simulink model "Microgrid_transition_model_113021_ben"  (R2020a)
settings: Solver=VariableStepAuto  StartTime=0.0  StopTime=1  MaxStep=1e-4  RelTol=1e-3
PreLoadFcn:
  | %run('FC_microgrid_param.m')
  | %load('gen_grid_init.mat')
InitFcn:
  | %load myisoModel_init;
  | run('FC_microgrid_param.m')
  | tic
  | run('CARTinitFcn.m')
  | %caseNo = 2;
  | 
  | %if (caseNo == 1)
  | %set_param(['Isolated_grid_paper_model_022521/SignalGen'], 'ActiveScenario', 'PStep222kW');
  | %else
  | %set_param(['Isolated_grid_paper_model_022521/SignalGen'], 'ActiveScenario', 'QStep222kVAr');
  | 
  | %end;
StopFcn:
  | toc
undefined symbols (not defined in the file or in its folder): breakpoints1, breakpoints2, cc_kp, cp_table_data, ctrl, D1, Delta, DiscIntNeverNeededParam, DT, FC_BESS, FC_PV_FirstSolar, find_system, gcbh, libFC_BESS, libFC_PV, LowerLimit, magnitude, oversize, pll_ki, pll_kp, pq_ts, sps_rtmsupport, timer, ts, Ts, Ts_APC, Ts_Control, Ts_Power, UpperLimit
libraries: powerlib x152, powerlib_extras x100, simulink x95, powerlib_meascontrol x90, eePowerMeasurement x40, pi_ctrl x16, simulink_extras x12, sps_avr x7, spsDieselMotorModel x3, libFSArray x2, SignalEditorBlockLib x2, libLgBattery x1
(part 1 of 14)
CloseFcn:
  | toc
settings Model: SimulationMode=accelerator  Creator=rpoudel  LastModifiedBy=banderso2
settings SolverCC: ZeroCrossAlgorithm=Adaptive
settings DataIOCC: SaveOperatingPoint=on  SaveFormat=StructureWithTime  SaveOutput=off  SignalLogging=off  DSMLogging=off  SaveTime=off  ReturnWorkspaceOutputs=off
settings OptimizationCC: EfficientMapNaN2IntZero=off
settings DebuggingCC: IgnoredZcDiagnostic=none  UnconnectedInputMsg=none  UnconnectedOutputMsg=none  UnconnectedLineMsg=none  ArithmeticOperatorsInVariantConditions=warning
settings HardwareCC: TargetBitPerPointer=64  TargetBitPerSizeT=64  TargetBitPerPtrDiffT=64  TargetLongLongMode=on  TargetIntDivRoundTo=Zero  TargetEndianess=LittleEndian  TargetWordSize=64  TargetHWDeviceType=MATLAB Host  ProdEqTarget=off
settings SFSimCC: SimUseLocalCustomCode=off  CustomCodeUndefinedFunction=UseInterfaceOnly
settings RTWCC: SystemTargetFile=accel.tlc  TemplateMakefile=accel_default_tmf  RTWVerbose=off
settings CodeAppCC: MaxIdLength=128
settings STFCustomTargetCC: TargetLangStandard=C99 (ISO)  ConcurrentExecutionCompliant=on  MATLABClassNameForMDSCustomization=Simulink.SoftwareTarget.TargetSpecificTriggerConfigurationBase  GRTInterface=on  SystemTargetFile=accel.tlc

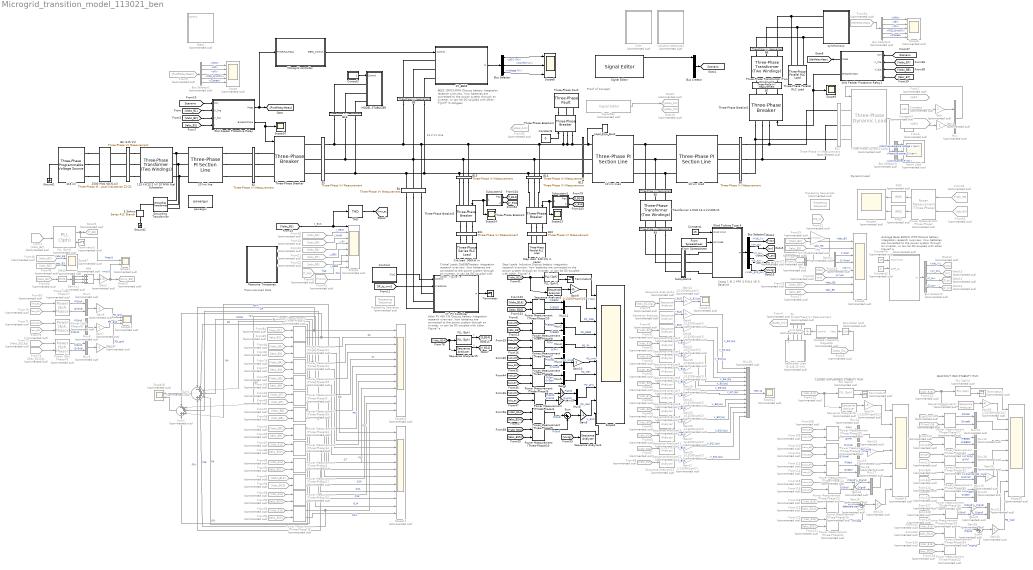
== system Microgrid_transition_model_113021_ben ==
  note: CLOSED UNPLANNED STABILITY RUN
  note: Dynamic Load
  note: Proof of Concept
  note: Critical Loads
      | Discuss battery integration research overview, how batteries are connected to the power system through an inverter, or can be DC-coupled with other. Figure?
      |
      | e
  note: Resource/Load Data
  note: 13.2 kV LIne
  note: Eaton Switchgear
  note: BESS 1MW/1MWh
      | Discuss battery integration research overview, how batteries are connected to the power system through an inverter, or can be DC-coupled with other. Figure?
      |
      | e
  note: Solar PV 430 kW
      | Discuss battery integration research overview, how batteries are connected to the power system through an inverter, or can be DC-coupled with other. Figure?
      |
      | e
  note: Step Loads: Inductive
      | Discuss battery integration research overview, how batteries are connected to the power system through an inverter, or can be DC-coupled with other. Figure?
      |
      | e
  note: Average Base 600kW WTG
      | Discuss battery integration research overview, how batteries are connected to the power system through an inverter, or can be DC-coupled with other. Figure?
      |
      | e
  note: Cases
      | 1 IR
      | 2 PFR
      | 3 P/Q
      | 4 VR
      | 5 Baseline
  note: BLACKOUT GEN STABILITY RUN
  .. : Subsystem  Commented=on  LoadFcn=%find_system(gcs,'FollowLinks', 'on', 'LookUnderMasks', 'all');  mask(Wind Turbine: Model 7){Nb_wt=1, ShowParameters=Drive train data for 1 wind turbine, nom=[6e5/0.9 730 60], Reactances=[ 1.305, 0.296, 0.252, 0.474,  0.243,  0.18 ], Time_constants=[4.49  0.0681  0.0513  ], Resistance=0.006, mec=[0.62/10 0.01 1], init=[ 0  0  0  0  0  0  0  0  1 ], Vnom=575, Imax_grid_conv=1.1, RL_grid=[ 0.15 0.15/50], C_var_filter1=150e3, Vdc_nom=1100, C_DClink1=90000e-6, L_R_Boost=[0.0012     5e-3], Pmec1=6e5, wind_speed_CpMax=11, wind0=11, DisplayTurbChar=off, H_WT=4.32, Ksh=0.0446, D_mutual=1.5, w_wt0=1, torque0=1, Kdc=[1.1   27.5], Ki_var_reg=0.05, Ki_volt_reg=2, Kgrid_side_cur_reg=[1  50], Kspeed=[5 1], Kboost_cur_reg=[0.025 100], Kp_pitch=15, Kcompensation=[1.5  6], Kfield=[10  20], pitch_max=27, pitch_rate=10, Ts=Ts}
      mask prompts: Nb_wt "Number of wind turbines:"; ShowParameters "Display:"; nom "Nom. power, L-L volt. and freq.: [Pn (VA), Vn (Vrms), fn (Hz)]"; Reactances "Reactances [Xd Xd' Xd'' Xq Xq'' Xl] (p.u.):"; Time_constants "Time constants [Tdo' Tdo'' Tq''] (s):"; Resistance "Resistance Rs (p.u.):"; mec "Inertia constant, friction factor, and pairs of poles: [ H(s)  F(p.u.)  p ]"; init "Initial conditions: [dw(%) th(deg) ia,ib,ic(pu) pha,phb,phc(deg) Vf(pu)]:"; Vnom "Grid-side converter nominal AC voltage (V):"; Imax_grid_conv "Grid-side converter maximum AC current (pu based on generator power and converter nominal AC voltage):"; RL_grid "Grid-side coupling inductor [ L(pu) R(pu),pu based on generator power and converter nominal AC voltage] :"; C_var_filter1 "Line filter capacitor (Q=50) (var):"; Vdc_nom "Nominal DC bus voltage (V)"; C_DClink1 "DC bus capacitor (F):"; L_R_Boost "Boost converter inductance [L(H) R(ohm)]:"; Pmec1 "Nominal mechanical output power (W):"; wind_speed_CpMax "Wind speed at nominal speed and at Cp max (must be between 6 m/s and 30 m/s) (m/s):"; wind0 "Initial wind speed (m/s):"; DisplayTurbChar "Display wind turbine power characteristics:"; H_WT "Wind turbine inertia constant H (s):"; Ksh "Shaft spring constant refer to high-speed shaft (pu of nominal mechanical torque/rad):"; D_mutual "Shaft mutual damping (pu of nominal mechanical torque/pu dw):"; w_wt0 "Turbine initial speed (pu of nominal speed):"; torque0 "Initial output torque (pu of nominal mechanical torque):"; Kdc "DC bus voltage regulator gains [Kp Ki]:"; Ki_var_reg "Grid-side converter var regulator gain [ Ki]:"; Ki_volt_reg "Grid-side converter voltage regulator gain [ Ki]:"; Kgrid_side_cur_reg "Grid-side converter current regulator gains [Kp Ki]:"; Kspeed "Speed regulator gains [Kp Ki]:"; Kboost_cur_reg "Boost inductor current regulator gains [Kp Ki]:"; Kp_pitch "Pitch controller gain [Kp]:"; Kcompensation "Pitch compensation gains [Kp Ki]:"; Kfield "Field excitation gains [Kp Ki]:"; pitch_max "Maximum pitch angle (deg):"; pitch_rate "Maximum rate of change of pitch angle (deg/s)"; Ts "Sample time (s):"
      mask help: This block implements a model of a variable speed pitch controlled wind turbine using a synchronous generator.
      mask init:
      | %Generator data
      | Pnom=nom(1)*Nb_wt;
      | Vnom_gen=nom(2);
      | Fnom=nom(3);
      | Xd=Reactances(1);
      | Xd1=Reactances(2);
      | Xd2=Reactances(3);
      | Xq=Reactances(4);
      | Xq2=Reactances(5);
      | Xl=Reactances(6);
      | Tdo1=Time_constants(1);
      | Tdo2=Time_constants(2);
      | Tq2=Time_constants(3);
      | H=mec(1);
      | F=mec(2);
      | p=mec(3);
      | 
      | % Converters data
      | L_RL=RL_grid(1);
      | R_RL=RL_grid(2);
      | L_Boost=L_R_Boost(1)/Nb_wt;
      | R_Boost=L_R_Boost(2)/Nb_wt;
      | Q_filter=50;
      | C_DClink=C_DClink1*Nb_wt;
      | C_var_filter=C_var_filter1*Nb_wt;
      | 
      | % Controller data
      | Freq_filter=10000;   %Hz
      | Zeta_filter=0.707;
      | Kp_dc=Kdc(1);
      | Ki_dc=Kdc(2);
      | Kp_grid_side_cur_reg=Kgrid_side_cur_reg(1);
      | Ki_grid_side_cur_reg=Kgrid_side_cur_reg(2);
      | Kp_speed=Kspeed(1);
      | Ki_speed=Kspeed(2);
      | Kp_boost_cur_reg=Kboost_cur_reg(1);
      | Ki_boost_cur_reg=Kboost_cur_reg(2);
      | Kp_compensation=Kcompensation(1);
      | Ki_compensation=Kcompensation(2);
      | Kp_field=Kfield(1);
      | Ki_field=Kfield(2);
      | Mod_index_max=1.1;
      | T_speed=5;      %Speed reference time constant (s)
      | Iq_ref_limit_time_constant=0.3; %(s)
      | Current_reg_output_limit=1.1;   %(pu)
      | Var_reg_output_hi_limit=1.1;    %(pu)
      | Var_reg_output_low_limit=0.9;   %(pu)
      | Pitch_time_constant=0.01;       %(s)
      | Vf_limit=10;    %Field voltage limit (pu)
      | Flux_meas_time_constant=1*(1/Fnom); %(s)
      | Ts_snub=50e-6;  %Sample time to compute snubber resistance
      | 
      | 
      | % Turbine data
      | Pmec=Pmec1*Nb_wt;
      | c1 = 0.6450;
      | c2 = 116;
      | c3 = .4;
      | c4 = 5;
      | c5 = 21;
      | c6 = .00912;  % Set Pmin in stall condition (does not vary with wind_speed_Pmax)
      | c7 = .08;
      | c8 = .035;
      | theta=0;
      | CpMax=.465;     %.5;
      | lambda_CpMax=6; %9.9495;
      | 
      | c1_c8=[c1 c2 c3 c4 c5 c6 c7 c8];
      |   
      | 
      | %   Cp = c1*(c6*lambda + (-c4 - c3*(2.5 + theta) + c2*(1/(lambda + ...
      | %   c7*(2.5 + theta)) - c8/(1 + (2.5 + theta)^3)))/exp(c5*(1/(lambda + ...
      | %   c7*(2.5 + theta)) - c8/(1 + (2.5 + theta)^3))))
      | 
      | 
      |         %%%%%%%%%%%%%%%%%%%%%%%%%%%%%%%%%%%%%%%%%%%%%%%%%%%%%%%%%%%%%%%%%%%%%%%%%%%
      |         % Operation at Cp max
      |         %%%%%%%%%%%%%%%%%%%%%%%%%%%%%%%%%%%%%%%%%%%%%%%%%%%%%%%%%%%%%%%%%%%%%%%%%%%
      |         
      |         rated_omegar=1;
      |         omegar = rated_omegar;
      |         
      |         % Enforce boundaries on wind speed
      |         % A warning could be displayed
      |         if wind_speed_CpMax < 6
      |             wind_speed_CpMax=6;
      |             disp('Warning: Wind speed at nominal speed and at Cp max has been set to 6 m/s')
      |         end
      |         if wind_speed_CpMax > 30
      |             wind_speed_CpMax=30;
      |             disp('Warning: Wind speed at nominal speed and at Cp max has been set to 30 m/s')
      |         end
      | 
      |         K1=lambda_CpMax/omegar*wind_speed_CpMax;
      |         
      |         % Calculation of K2 needed to get P equal to the requested value at
      |         % Cp max for the requested wind speed
      |         
      |         Prated=Pmec;
      |         P_rated_omegar_theta_zero=1; %0.75;
      |         
      |         K2 = P_rated_omegar_theta_zero*Prated/(wind_speed_CpMax^3*CpMax);
      |         
      |         K1_K2=[K1 K2];
      |         
      |         %%%%%%%%%%%%%%%%%%%%%%%%%%%%%%%%%%%%%%%%%%%%%%%%%%%%%%%%%%%%%%%%%%%%%%%%%%%
      |         % End of calculation for operation at Cp max
      |         %%%%%%%%%%%%%%%%%%%%%%%%%%%%%%%%%%%%%%%%%%%%%%%%%%%%%%%%%%%%%%%%%%%%%%%%%%%
      |         
      | 
      | %%%%%%%%%%%%%%%%%%%%%%%%%%%%%%%%%%%%%%%%%%%%%%%%%%%%%%%%%%%%%%%%%%%%%%%%%%%
      | % Plot turbine characteristics
      | %%%%%%%%%%%%%%%%%%%%%%%%%%%%%%%%%%%%%%%%%%%%%%%%%%%%%%%%%%%%%%%%%%%%%%%%%%% 
      | 
      | DisplayTurbChar=get_param(gcb,'DisplayTurbChar');
      | if strcmp(DisplayTurbChar,'on')
      |     vect_theta = 0:2:30;
      |     
      |     vect_lambda = 1:0.2:30;
      |     
      |     clear Cp;
      |     
      |     for i=1:length(vect_theta)
      |      for j=1:length(vect_lambda)
      |                 Cp(i,j) = c1*(c6*vect_lambda(j) + (-c4 - c3*(2.5 + vect_theta(i)) + c2*(1/(vect_lambda(j) + ...
      |                 c7*(2.5 + vect_theta(i))) - c8/(1 + (2.5 + vect_theta(i))^3)))/exp(c5*(1/(vect_lambda(j) + ...
      |                 c7*(2.5 + vect_theta(i))) - c8/(1 + (2.5 + vect_theta(i))^3))));
      |      end
      |     end
      | 
      |     figure(1);
      |     clf;
      |     hold on;
      | 
      |     plot(vect_lambda, Cp);
      |     axis([0, 25, 0, .6]);
      |     title('Wind Turbine Cp Characteristic (pitch angle increases by step of 2 deg.)');
      |     ylabel('Cp');
      |     set(gca,'ytick',[0 .1 .2 .3 .4 .5 .6]);
      |     xlabel('Lambda');
      |     grid on;
      |     text(10.1,0.51,'Pitch angle 0 degree');
      | 
      |     hold off
      |     
      |     % Plot of the wind turbine mechanical power output (pu) lambda and Cp
      |     % characteristics against wind speed (m/s) for a range of theta.
      |     
      |     wind_speed_range = [1,.2,30];
      |     vect_wind_speed = 1:0.2:30;
      |     
      |     clear lambda;
      |     clear Cp;
      |     clear P;
      | 
      |     for i=1:length(vect_theta)
      |         for j=1:length(vect_wind_speed)
      |             lambda(i,j) = K1*omegar/vect_wind_speed(j);
      |             Cp(i,j) = c1*(c6*lambda(i,j) + (-c4 - c3*(2.5 + vect_theta(i)) + c2*(1/(lambda(i,j) + ...
      |             c7*(2.5 + vect_theta(i))) - c8/(1 + (2.5 + vect_theta(i))^3)))/exp(c5*(1/(lambda(i,j) + ...
      |             c7*(2.5 + vect_theta(i))) - c8/(1 + (2.5 + vect_theta(i))^3))));
      |             P(i,j) = K2/Prated*vect_wind_speed(j)^3*Cp(i,j);
      |         end
      |     end
      |     
      |     
      |     figure(2);
      |     clf;
      |     hold on
      |     
      |     subplot(3,1,1);
      |     plot(vect_wind_speed, P);
      |     axis([0, 35, 0, 1.5]);
      |     title('Wind Turbine Characteristics (w = 1 pu, pitch angle increases by step of 2 deg.)');
      |     ylabel('P (pu)');
      |     set(gca,'ytick',0:.5:4);
      |     grid on;
      |     
      |     subplot(3,1,2);
      |     plot(vect_wind_speed, lambda);
      |     axis([0, 35, 0, 20]);
      |     ylabel('Lambda');
      |     grid on;
      |     
      |     subplot(3,1,3)
      |     plot(vect_wind_speed, Cp);
      |     axis([0, 35, 0, .6]);
      |     xlabel('Wind Speed (m/s)');
      |     ylabel('Cp');
      |     set(gca,'ytick',[0 .1 .2 .3 .4 .5 .6]);
      |     grid on;
      | 
      |     hold off
      |     set_param(gcb,'DisplayTurbChar','off')
      |     
      | end
      mask TypeOptions ShowParameters: Generator data for 1 wind turbine | Converters data for 1 wind turbine | Turbine data for 1 wind turbine | Drive train data for 1 wind turbine | Control parameters for 1 wind turbine
      mask Callback ShowParameters:
      | BlockName=getfullname(gcb);
      | %
      | Param_Show=get_param(BlockName,'ShowParameters');
      | Param_DisplayTurbChar=get_param(BlockName,'DisplayTurbChar');
      | 
      | p_mask{3}='off';p_mask{4}='off';p_mask{5}='off';
      | p_mask{6}='off';p_mask{7}='off';p_mask{8}='off';p_mask{9}='off';
      | p_mask{10}='off';p_mask{11}='off';p_mask{12}='off';p_mask{13}='off';
      | p_mask{14}='off';p_mask{15}='off';p_mask{16}='off';p_mask{17}='off';
      | p_mask{18}='off';p_mask{19}='off';p_mask{20}='off';p_mask{21}='off';
      | p_mask{22}='off';p_mask{23}='off';p_mask{24}='off';p_mask{25}='off';
      | p_mask{26}='off';p_mask{27}='off';p_mask{28}='off';p_mask{29}='off';
      | p_mask{30}='off';p_mask{31}='off';p_mask{32}='off';p_mask{33}='off';
      | p_mask{34}='off';p_mask{35}='off';
      | 
      | switch Param_Show
      | 	case 'Generator data for 1 wind turbine'
      | 		p_mask{3}='on';p_mask{4}='on';p_mask{5}='on';
      |         p_mask{6}='on';p_mask{7}='on';p_mask{8}='on';
      |     case 'Converters data for 1 wind turbine'
      | 		p_mask{9}='on';p_mask{10}='on';p_mask{11}='on';
      |         p_mask{12}='on';p_mask{13}='on';p_mask{14}='on';p_mask{15}='on';
      | 	case 'Turbine data for 1 wind turbine'
      | 		p_mask{16}='on';p_mask{17}='on';p_mask{18}='on';p_mask{19}='on';
      |     case 'Drive train data for 1 wind turbine'
      |         p_mask{20}='on';p_mask{21}='on';p_mask{22}='on';p_mask{23}='on';
      |         p_mask{24}='on';
      |     case 'Control parameters for 1 wind turbine'
      |         p_mask{25}='on';p_mask{26}='on';p_mask{27}='on';
      |         p_mask{28}='on';p_mask{29}='on';p_mask{30}='on';p_mask{31}='on';
      |         p_mask{32}='on';p_mask{33}='on';p_mask{34}='on';p_mask{35}='on';
      | end
      | 
      | ParVisible={'on','on',p_mask{3},p_mask{4},p_mask{5},p_mask{6},...
      |     p_mask{7},p_mask{8},p_mask{9},p_mask{10},p_mask{11},p_mask{12},...
      |     p_mask{13},p_mask{14},p_mask{15},p_mask{16},p_mask{17},p_mask{18},...
      |     p_mask{19},p_mask{20},p_mask{21},p_mask{22},p_mask{23},p_mask{24},...
      |     p_mask{25},p_mask{26},p_mask{27},p_mask{28},p_mask{29},p_mask{30},...
      |     p_mask{31},p_mask{32},p_mask{33},p_mask{34},p_mask{35},'on'};
      | %
      | set_param(BlockName,'MaskVisibilities',ParVisible);
      | set_param(BlockName,'DisplayTurbChar',Param_DisplayTurbChar);
      mask Display: image('$imagefile'); % Use "Edit Image" on toolstrip to change.
  10 km line : powerlib/Elements/Three-Phase PI Section Line  LConnTagsString=a|b|c  RConnTagsString=A|B|C  Frequency=60  Resistances=[0.1153 0.413]  Inductances=[1.05e-3 3.32e-3]  Capacitances=[11.33e-009 5.01e-009]  Length=10
  10 km line1 : powerlib/Elements/Three-Phase PI Section Line  LConnTagsString=a|b|c  RConnTagsString=A|B|C  Frequency=60  Resistances=[0.1153 0.413]  Inductances=[1.05e-3 3.32e-3]  Capacitances=[11.33e-009 5.01e-009]  Length=0.1
  10 km line2 : powerlib/Elements/Three-Phase PI Section Line  LConnTagsString=a|b|c  RConnTagsString=A|B|C  Frequency=60  Resistances=[0.1153 0.413]  Inductances=[1.05e-3 3.32e-3]  Capacitances=[11.33e-009 5.01e-009]  Length=0.01
  115 kV : powerlib/Electrical Sources/Three-Phase Programmable Voltage Source  PositiveSequence=[115e3 0 60]  VariationEntity=None  VariationType=Table of time-amplitude pairs  VariationTypeAlt=Step  VariationStep=-0.2  VariationRate=10  VariationMagnitude=0.3  VariationFrequency=2  VariationTiming=[0.05 0.05+5/60]  VariationPhaseA=off  Amplitudes=[1 1 1.0]  TimeValues=[0 0.03 0.13]  HarmonicGeneration=off  HarmonicA=[1 -0.1 0 2]  HarmonicB=[2 0.15 35 2]*0  Timing="[0.1  2]"  BusType=swing  Pref=0  Qref=0  Qmin=-inf  Qmax=inf
  115 kV/13.2 kV 10 MVA Xcel Substation : powerlib/Elements/Three-Phase Transformer (Two Windings)  Winding1Connection=Yg  Winding2Connection=Delta (D1)  CoreType=Three single-phase transformers  SetSaturation=off  Hysteresis=off  DataFile='basic_model'  SetInitialFlux=off  Measurements=None  UNITS=pu  NominalPower=[10e6 60 ]  Winding1="[ 115e3  0.08/30   0.08 ]"  Winding2="[ 13.2e3  0.08/30  0.08]"  Rm=500  Lm=500  L0=0.5  Saturation="[ 0,0  ;  0.005,1.2  ;  1.0,1.4 ]"  InitialFluxes=[ 0.8 , -0.8 , 0.7 ]  BreakLoop=off  DiscreteSolver=Trapezoidal iterative  DataType=off  TransfoNumber=0
  2500 MVA X0/X1=3 : powerlib/Elements/Three-Phase Mutual Inductance Z1-Z0  LConnTagsString=a|b|c  RConnTagsString=A|B|C  PositiveSequence="[0.1  1.0/(2*pi*60)] *115e3^2/2500e6"  ZeroSequence="[0.3  3.0/(2*pi*60)] *115e3^2/2500e6"
      settings: SourceProductBaseCode=PS
  "3.3ohms " : powerlib/Elements/Series RLC Branch  LConnTagsString=__new0  RConnTagsString=__new0  BranchType=R  Resistance=3.3  Inductance=[]  SetiL0=off  InitialCurrent=0  Capacitance=[]  Setx0=off  InitialVoltage=0  Measurements=None
  Active Load : Scope  Commented=on  NumInputPorts=3
  Add : Sum  Commented=on  Inputs=+++
  B1 : powerlib/Measurements/Three-Phase V-I Measurement  VoltageMeasurement=phase-to-ground  SetLabelV=on  LabelV=Vabc_B1  Vpu=off  VpuLL=off  CurrentMeasurement=yes  SetLabelI=on  LabelI=Iabc_B1  Ipu=off  Pbase=100e6  Vbase=440  OutputType=Magnitude  PhasorSimulation=off  PSBequivalent=0
  B10 : powerlib/Measurements/Three-Phase V-I Measurement  VoltageMeasurement=phase-to-ground  SetLabelV=on  LabelV=Vabc_B10  Vpu=off  VpuLL=off  CurrentMeasurement=yes  SetLabelI=on  LabelI=Iabc_B10  Ipu=off  Pbase=100e6  Vbase=440  OutputType=Magnitude  PhasorSimulation=off  PSBequivalent=0
  B11 : powerlib/Measurements/Three-Phase V-I Measurement  VoltageMeasurement=phase-to-ground  SetLabelV=on  LabelV=Vabc_B11  Vpu=off  VpuLL=off  CurrentMeasurement=yes  SetLabelI=on  LabelI=Iabc_B11  Ipu=off  Pbase=100e6  Vbase=440  OutputType=Magnitude  PhasorSimulation=off  PSBequivalent=0
  B12 : powerlib/Measurements/Three-Phase V-I Measurement  Commented=on  VoltageMeasurement=phase-to-ground  SetLabelV=on  LabelV=Vabc_B12  Vpu=off  VpuLL=off  CurrentMeasurement=yes  SetLabelI=on  LabelI=Iabc_B12  Ipu=off  Pbase=100e6  Vbase=440  OutputType=Magnitude  PhasorSimulation=off  PSBequivalent=0
  B13 : powerlib/Measurements/Three-Phase V-I Measurement  VoltageMeasurement=phase-to-ground  SetLabelV=on  LabelV=Vabc_B13  Vpu=off  VpuLL=off  CurrentMeasurement=yes  SetLabelI=on  LabelI=Iabc_B13  Ipu=off  Pbase=100e6  Vbase=440  OutputType=Magnitude  PhasorSimulation=off  PSBequivalent=0
  B14 : powerlib/Measurements/Three-Phase V-I Measurement  VoltageMeasurement=phase-to-ground  SetLabelV=on  LabelV=Vabc_B14  Vpu=off  VpuLL=off  CurrentMeasurement=yes  SetLabelI=on  LabelI=Iabc_B14  Ipu=off  Pbase=100e6  Vbase=440  OutputType=Magnitude  PhasorSimulation=off  PSBequivalent=0
  B15 : powerlib/Measurements/Three-Phase V-I Measurement  VoltageMeasurement=phase-to-ground  SetLabelV=on  LabelV=Vabc_B15  Vpu=off  VpuLL=off  CurrentMeasurement=yes  SetLabelI=on  LabelI=Iabc_B15  Ipu=off  Pbase=100e6  Vbase=440  OutputType=Magnitude  PhasorSimulation=off  PSBequivalent=0
  B16 : powerlib/Measurements/Three-Phase V-I Measurement  VoltageMeasurement=phase-to-ground  SetLabelV=on  LabelV=Vabc_B16  Vpu=off  VpuLL=off  CurrentMeasurement=yes  SetLabelI=on  LabelI=Iabc_B16  Ipu=off  Pbase=100e6  Vbase=440  OutputType=Magnitude  PhasorSimulation=off  PSBequivalent=0
  B2 : powerlib/Measurements/Three-Phase V-I Measurement  VoltageMeasurement=phase-to-ground  SetLabelV=on  LabelV=Vabc_B2  Vpu=off  VpuLL=off  CurrentMeasurement=yes  SetLabelI=on  LabelI=Iabc_B2  Ipu=off  Pbase=100e6  Vbase=440  OutputType=Magnitude  PhasorSimulation=off  PSBequivalent=0
  B3 : powerlib/Measurements/Three-Phase V-I Measurement  VoltageMeasurement=phase-to-ground  SetLabelV=on  LabelV=Vabc_B3  Vpu=off  VpuLL=off  CurrentMeasurement=yes  SetLabelI=on  LabelI=Iabc_B3  Ipu=off  Pbase=618460*oversize  Vbase=575  OutputType=Magnitude  PhasorSimulation=off  PSBequivalent=0
  B3 (115 kV) : powerlib/Measurements/Three-Phase V-I Measurement  VoltageMeasurement=phase-to-ground  SetLabelV=on  LabelV=Vabc_B115g  Vpu=off  VpuLL=off  CurrentMeasurement=yes  SetLabelI=on  LabelI=Iabc_B115g  Ipu=off  Pbase=100e6  Vbase=120e3  OutputType=Complex  PhasorSimulation=off  PSBequivalent=0
  B4 : powerlib/Measurements/Three-Phase V-I Measurement  VoltageMeasurement=phase-to-ground  SetLabelV=on  LabelV=Vabc_B4  Vpu=off  VpuLL=off  CurrentMeasurement=yes  SetLabelI=on  LabelI=Iabc_B4  Ipu=off  Pbase=100e6  Vbase=440  OutputType=Magnitude  PhasorSimulation=off  PSBequivalent=0
  B5 : powerlib/Measurements/Three-Phase V-I Measurement  VoltageMeasurement=phase-to-ground  SetLabelV=on  LabelV=Vabc_B5  Vpu=off  VpuLL=off  CurrentMeasurement=yes  SetLabelI=on  LabelI=Iabc_B5  Ipu=off  Pbase=100e6  Vbase=440  OutputType=Magnitude  PhasorSimulation=off  PSBequivalent=0
  B6 : powerlib/Measurements/Three-Phase V-I Measurement  VoltageMeasurement=phase-to-ground  SetLabelV=on  LabelV=Vabc_B6  Vpu=off  VpuLL=off  CurrentMeasurement=yes  SetLabelI=on  LabelI=Iabc_B6  Ipu=off  Pbase=100e6  Vbase=440  OutputType=Magnitude  PhasorSimulation=off  PSBequivalent=0
  B7 : powerlib/Measurements/Three-Phase V-I Measurement  VoltageMeasurement=phase-to-ground  SetLabelV=on  LabelV=Vabc_B7  Vpu=off  VpuLL=off  CurrentMeasurement=yes  SetLabelI=on  LabelI=Iabc_B7  Ipu=off  Pbase=100e6  Vbase=440  OutputType=Magnitude  PhasorSimulation=off  PSBequivalent=0
  B8 : powerlib/Measurements/Three-Phase V-I Measurement  VoltageMeasurement=phase-to-ground  SetLabelV=on  LabelV=Vabc_B8  Vpu=off  VpuLL=off  CurrentMeasurement=yes  SetLabelI=on  LabelI=Iabc_B8  Ipu=off  Pbase=100e6  Vbase=440  OutputType=Magnitude  PhasorSimulation=off  PSBequivalent=0
  B9 : powerlib/Measurements/Three-Phase V-I Measurement  VoltageMeasurement=phase-to-ground  SetLabelV=on  LabelV=Vabc_B9  Vpu=off  VpuLL=off  CurrentMeasurement=yes  SetLabelI=on  LabelI=Iabc_B9  Ipu=off  Pbase=100e6  Vbase=440  OutputType=Magnitude  PhasorSimulation=off  PSBequivalent=0
  Bus Creator : BusCreator  Inputs=7
  Bus Selector : BusSelector  OutputSignals=SOC (%),Current (A),Voltage (V)
  Bus Selector1 : BusSelector  Commented=on  OutputSignals=R25_Meas.dWt,R25_Meas.dF,R25_Meas.dV,R25_SyncOK,Closed
  Bus Selector2 : BusSelector  OutputSignals=Vdc_V,wr_pu,PQ_pu.P_pu,PQ_pu.Q_pu,Vabc_grid_pu
  Bus Selector3 : BusSelector  Commented=on  OutputSignals=Positive-sequence voltage V (pu),Reactive power Q (var),Active power P (W)
  Bus Selector4 : BusSelector  Commented=on  OutputSignals=R25_Meas.dWt,R25_Meas.dF,R25_Meas.dV,R25_SyncOK,Closed
  Bus Selector5 : BusSelector  Commented=on  OutputSignals=Vdc_V,wr_pu,PQ_pu.P_pu,PQ_pu.Q_pu
  Constant : Constant  Commented=on  Value=130
  Constant1 : Constant  Value=15
  Constant2 : Constant  Commented=on  Value=0
  Constant3 : Constant  Value=0
  Constant4 : Constant  Commented=on  Value=15
  Constant7 : Constant  Commented=on  Value=30
  Control1 : Subsystem
  Control3 : Subsystem
  Crit load. 900kW in paper : powerlib/Elements/Three-Phase Series RLC Load  LConnTagsString=A|B|C  Configuration=Y (grounded)  NominalVoltage=13.2e3  Vabc=[1e3 1e3 1e3]  Vabcp=[1e3 1e3 1e3]  NominalFrequency=60  UnbalancedPower=off  ActivePower=15e5  InductivePower=0  CapacitivePower=0  Pabc=[10e3 9e3 11e3]  QLabc=[100 90 110]  QCabc=[100 90 110]  Pabcp=[10e3 9e3 11e3]  QLabcp=[100 90 110]  QCabcp=[100 90 110]  Measurements=None  LoadType=constant Z
  Defferable Load (0-446.25 kW) : Subsystem  Commented=on  mask(8-step Variable Load){Vphase_phase_lissage=13200*sqrt(2/3), Freq=60, P_lissage_min=1.75e3, Pin_3phase=50e3}
      mask prompts: Vphase_phase_lissage "Nominal L-L voltage (Vrms):"; Freq "Nominal frequency (Hz):"; P_lissage_min "Power per step Pstep (W):"; Pin_3phase "Initial power  (W) :"
      mask help:
      | This block implements a variable, three-phase resistive load. The load variation uses an eight-bit binary progression so that the load power can be varied by steps from 0 to 255*Pstep.
      |
      | The eight three-phase resistors are connected in series with ideal switches simulating forced-commutated power electronic switches.
      |
      | The Pulses input is a vector containing the eight bits (0/1) controlling the eight three-phase switches. First value is the less significant bit.
      mask init:
      | Ron_switch=1e-6;
      | Rs_snubber=inf;
      | Cs_snubber=0;
      | n_niveaux=8;
      | Pmax=((2^n_niveaux)-1)*P_lissage_min;
      | Pin_normalise=min([(Pin_3phase/Pmax)*((2^n_niveaux)-1) ((2^n_niveaux)-1)]);
      | discret1=pow2(0:-1:-(n_niveaux-1))*Pin_normalise;
      | discret2=floor(discret1);
      | Status=rem(discret2,2);
  Demux : Demux  Commented=on  Outputs=2
  Demux1 : Demux  Commented=on  Outputs=3
  Discrete Frequency Regulator : Subsystem  Commented=on  mask(Discrete Frequency Regulator){Freq_ref=60, gains_regulator=[255 30], Vpp_nom=13200, Ts=Ts}
      mask prompts: Freq_ref "Reference frequency (Hz):"; gains_regulator "Regulator gains  [Kp Kd]:"; Vpp_nom "Phase to phase voltage (Vrms):"; Ts "Sample time (s):"
      mask help:
      | Input : phase to ground voltages
      |
      | Output : 24 logical signals for the control of the dump load
      mask init:
      | Vbase=Vpp_nom/sqrt(3);
      | Kp=gains_regulator(1);
      | Kd=gains_regulator(2);
  FC_BESS : Subsystem  AncestorBlock=libFC_BESS/FC_BESS  mask{EnBattery=on, Ts=Ts, cc_kp=-1, cc_Ti=-1, pll_kp=-1, pll_ki=-1}
      mask prompts: EnBattery "Enable Battery Model"; Ts "Sampling time"; cc_kp "Current Controller - kp [pu]"; cc_Ti "Current Controller - Ti [s]"; pll_kp "PLL - kp [pu]"; pll_ki "PLL - ki [pu]"
      mask DialogControl Generaltab Prompt: General
      mask DialogControl InverterTuningTab Prompt: Tuning
      mask DialogControl Control2 Prompt: Use -1 to use default validate SMA inverter values
      mask Display: image('$imagefile'); % Use "Edit Image" on toolstrip to change.
  FC_PV_FirstSolar : Subsystem  AncestorBlock=libFC_PV/FC_PV_FirstSolar  mask{EnArray=on, Ts=Ts, cc_kp=-1, cc_Ti=-1, pll_kp=-1, pll_ki=-1}
      mask prompts: EnArray "Enable Array Model"; Ts "Sampling time"; cc_kp "Current Controller - kp [pu]"; cc_Ti "Current Controller - Ti [s]"; pll_kp "PLL - kp [pu]"; pll_ki "PLL - ki [pu]"
      mask DialogControl Generaltab Prompt: General
      mask DialogControl InverterTuningTab Prompt: Tuning
      mask DialogControl Control2 Prompt: Use -1 to use default validate SMA inverter values
      mask Display: image('$imagefile'); % Use "Edit Image" on toolstrip to change.
  From Spreadsheet : FromSpreadsheet  FileName=Microgrid_cmd.xlsx  SheetName=WTGmode  SampleTime=-1
  From{1,25,48,50,52,80,110,123} (8 alike) : From  Commented=on  GotoTag=Vabc_B3  TagVisibility=global
      From25 settings: CloseFcn=tagdialog Close
      From48 settings: CloseFcn=tagdialog Close
      From50 settings: CloseFcn=tagdialog Close
  From100 : From  Commented=on  GotoTag=Iabc_B5  TagVisibility=global
  From105 : From  Commented=on  GotoTag=Iabc_B16  TagVisibility=global
  From106 : From  Commented=on  GotoTag=Vabc_B16  TagVisibility=global
  From107 : From  Commented=on  GotoTag=Iabc_B9  TagVisibility=global
  From{60,76,108,117} (4 alike) : From  Commented=on  GotoTag=Vabc_B4  TagVisibility=global
  From{20,77,109,122} (4 alike) : From  Commented=on  GotoTag=Iabc_B4  TagVisibility=global
  From{26,49,81,111,124} (5 alike) : From  Commented=on  GotoTag=Iabc_B3  TagVisibility=global
      From26 settings: CloseFcn=tagdialog Close
      From49 settings: CloseFcn=tagdialog Close
  From112 : From  Commented=on  GotoTag=Vabc_B13  TagVisibility=global
  From{63,82,113,126} (4 alike) : From  Commented=on  GotoTag=Vabc_B7  TagVisibility=global
  From{21,83,114,127} (4 alike) : From  Commented=on  GotoTag=Iabc_B7  TagVisibility=global
  From{40,69,84,115,128} (5 alike) : From  Commented=on  GotoTag=Vabc_B1  TagVisibility=global
  From{18,70,85,116,129} (5 alike) : From  Commented=on  GotoTag=Iabc_B1  TagVisibility=global
  From118 : From  Commented=on  GotoTag=Vabc_B14  TagVisibility=global
  From119 : From  Commented=on  GotoTag=Iabc_B14  TagVisibility=global
  From12 : From  Commented=on  GotoTag=WS_ts  TagVisibility=global
  From120 : From  Commented=on  GotoTag=Vabc_B15  TagVisibility=global
  From121 : From  Commented=on  GotoTag=Iabc_B15  TagVisibility=global
  From125 : From  Commented=on  GotoTag=Vabc_B13  TagVisibility=global
  From131 : From  Commented=on  GotoTag=Vabc_B14  TagVisibility=global
  From132 : From  Commented=on  GotoTag=Iabc_B14  TagVisibility=global
  From133 : From  Commented=on  GotoTag=Vabc_B15  TagVisibility=global
  From134 : From  Commented=on  GotoTag=Iabc_B15  TagVisibility=global
  From135 : From  Commented=on  GotoTag=Vabc_B9  TagVisibility=global
  From17 : From  Commented=on  GotoTag=Iabc_B5  TagVisibility=global
      settings: CloseFcn=tagdialog Close
  From19 : From  Commented=on  GotoTag=Iabc_B5  TagVisibility=global
  From2 : From  Commented=on  GotoTag=VARP  TagVisibility=global
  From22 : From  Commented=on  GotoTag=Iabc_B9  TagVisibility=global
  From23 : From  Commented=on  GotoTag=Vdc
      settings: CloseFcn=tagdialog Close
  From24 : From  Commented=on  GotoTag=wr
      settings: CloseFcn=tagdialog Close
  From27 : From  Commented=on  GotoTag=Q_pu
      settings: CloseFcn=tagdialog Close
  From28 : From  Commented=on  GotoTag=P_pu
      settings: CloseFcn=tagdialog Close
  From29 : From  Commented=on  GotoTag=Vabc_B5  TagVisibility=global
      settings: CloseFcn=tagdialog Close
  From32 : From  Commented=on  GotoTag=Vabc_B6  TagVisibility=global
  From33 : From  Commented=on  GotoTag=Iabc_B6  TagVisibility=global
  From34 : From  Commented=on  GotoTag=GenRelayMeas
  From35 : From  Commented=on  GotoTag=qstep_brk
  From4 : From  Commented=on  GotoTag=pstep_brk
  From42 : From  Commented=on  GotoTag=f_cgi
  From43 : From  Commented=on  GotoTag=THD_B1
  From5 : From  Commented=on  GotoTag=Vabc_SL  TagVisibility=global
      settings: CloseFcn=tagdialog Close
  From51 : From  Commented=on  GotoTag=Vabc_B2  TagVisibility=global
  From55 : From  Commented=on  GotoTag=Iabc_B9  TagVisibility=global
  From6 : From  Commented=on  GotoTag=VARQ  TagVisibility=global
  From61 : From  Commented=on  GotoTag=Vabc_B5  TagVisibility=global
  From62 : From  Commented=on  GotoTag=Vabc_B6  TagVisibility=global
  From64 : From  Commented=on  GotoTag=Vabc_B8  TagVisibility=global
  From65 : From  Commented=on  GotoTag=Vabc_B9  TagVisibility=global
  From66 : From  Commented=on  GotoTag=Vabc_B10  TagVisibility=global
  From67 : From  Commented=on  GotoTag=Vabc_B11  TagVisibility=global
  From68 : From  Commented=on  GotoTag=Vabc_B12
  From71 : From  Commented=on  GotoTag=Vabc_B2  TagVisibility=global
  From72 : From  Commented=on  GotoTag=Iabc_B2  TagVisibility=global
  From73 : From  Commented=on  GotoTag=Vabc_B115g  TagVisibility=global
  From74 : From  Commented=on  GotoTag=Iabc_B115g  TagVisibility=global
  From75 : From  Commented=on  GotoTag=Vabc_B115g  TagVisibility=global
  From86 : From  Commented=on  GotoTag=Vabc_B14  TagVisibility=global
  From87 : From  Commented=on  GotoTag=Vabc_B10  TagVisibility=global
  From88 : From  Commented=on  GotoTag=Iabc_B10  TagVisibility=global
  From89 : From  Commented=on  GotoTag=Vabc_B11  TagVisibility=global
  From9 : From  Commented=on  GotoTag=ProtRelayMeas
  From90 : From  Commented=on  GotoTag=Iabc_B11  TagVisibility=global
  From91 : From  Commented=on  GotoTag=Vabc_B9  TagVisibility=global
  From92 : From  Commented=on  GotoTag=Iabc_B14  TagVisibility=global
  From93 : From  Commented=on  GotoTag=Vabc_B15  TagVisibility=global
  From94 : From  Commented=on  GotoTag=Iabc_B15  TagVisibility=global
  From95 : From  Commented=on  GotoTag=Vabc_B13  TagVisibility=global
  From96 : From  Commented=on  GotoTag=Iabc_B13  TagVisibility=global
  From97 : From  Commented=on  GotoTag=Vabc_B8  TagVisibility=global
  From98 : From  Commented=on  GotoTag=Iabc_B8  TagVisibility=global
  From99 : From  Commented=on  GotoTag=Vabc_B5  TagVisibility=global
  Gain{,1,13,26} (4 alike) : Gain  Commented=on
  Gain10 : Gain
  Gain11 : Gain  Commented=on  Gain=1/575/sqrt(2)
  Gain{5,7,12,16,20,22,28,30,32} (9 alike) : Gain  Commented=on  Gain=-1
  Gain14 : Gain  Commented=on  Gain=1/115000/sqrt(2)
  Gain{6,8,15,17,21,23,25,27,29,31} (10 alike) : Gain  Commented=on  Gain=1/13200/sqrt(2)
  Gain18 : Gain  Gain=-1
  Gain19 : Gain  Commented=on  Gain=1/460/sqrt(2)
  Gain2 : Gain  Commented=on  Gain=1/3
  Gain24 : Gain  Commented=on  Gain=1/13200*sqrt(3/2)
  Gain3 : Gain  Gain=-1
  Gain33 : Gain  Commented=on  Gain=1/13200*sqrt(3/2)
  Gain4 : Gain  Gain=-1
  Gain9 : Gain  Gain=1/13200*sqrt(3/2)
  Goto10 : Goto  Commented=on  GotoTag=qstep_brk
  Goto11 : Goto  Commented=on  GotoTag=P_pu
  Goto12 : Goto  Commented=on  GotoTag=Vdc
  Goto13 : Goto  Commented=on  GotoTag=wr
  Goto14 : Goto  Commented=on  GotoTag=Q_pu
  Goto19 : Goto  Commented=on  GotoTag=f_B3
  Goto20 : Goto  Commented=on  GotoTag=Vrms_B3
  Goto9 : Goto  Commented=on  GotoTag=pstep_brk
  Grid Feeder Protective Relay : Subsystem
  Grid Feeder Protective Relay1 : Subsystem
  Ground1 : powerlib/Elements/Ground  LConnTagsString=a
  Ground2 : powerlib/Elements/Ground  LConnTagsString=a
  "Grounding Transformer " : powerlib/Elements/Grounding Transformer   UNITS=pu  NominalPower="[100e6   60]"  NominalVoltage=25e3  ZeroSequenceImpedance_pu=[0.025 0.75]  MagnetizationBranch_pu=[500 500]  ZeroSequenceImpedance_SI=[0.052083 589.05]  MagnetizationBranch_SI=[1041.7 3.927e+005]  Measurements=None
      settings: SourceProductBaseCode=PS
  Load Flow Bus2 : powerlib/Measurements/Load Flow Bus  LConnTagsString=a  Phases=single  Connectors=on one side  ID=BUS_1  Vbase=13.2e3  Vref=1  Vangle=0  VLF=1  VLFb=1  VLFc=1  angleLF=0  angleLFb=0  angleLFc=0
  MODEL STABILIZER : Subsystem  AncestorBlock=libFC_PV/FC_PV_FirstSolar  mask{EnArray=on, Ts=Ts, cc_kp=-1, cc_Ti=-1, pll_kp=-1, pll_ki=-1}
      mask prompts: EnArray "Enable Array Model"; Ts "Sampling time"; cc_kp "Current Controller - kp [pu]"; cc_Ti "Current Controller - Ti [s]"; pll_kp "PLL - kp [pu]"; pll_ki "PLL - ki [pu]"
      mask DialogControl Generaltab Prompt: General
      mask DialogControl InverterTuningTab Prompt: Tuning
      mask DialogControl Control2 Prompt: Use -1 to use default validate SMA inverter values
  MW : Gain  Commented=on  Gain=1*0.6/0.9  SaturateOnIntegerOverflow=on  OutDataTypeStr=Inherit: Same as input  ParamDataTypeStr=Inherit: Same as input
  Microgrid controller : Subsystem
  Mux{,1,7..9,12..21} (15 alike) : Mux  Commented=on  Inputs=2
  Mux10 : Mux  Commented=on  Inputs=12
  Mux{2..6,11} (6 alike) : Mux  Inputs=2
  PLL (3ph) : powerlib_meascontrol/PLL/PLL (3ph)  Fmin=45  Par_Init=[0, 60]  ParK=[180, 3200, 1]  TcD=1e-4  MaxRateChangeFreq=12  FilterCutOffFreq=25  Ts=0  AGC=on
  PLL (3ph)1 : powerlib_meascontrol/PLL/PLL (3ph)  Fmin=45  Par_Init=[0, 60]  ParK=[180, 3200, 1]  TcD=1e-4  MaxRateChangeFreq=12  FilterCutOffFreq=25  Ts=0  AGC=on
  PLL (3ph)2 : powerlib_meascontrol/PLL/PLL (3ph)  Commented=on  Fmin=45  Par_Init=[0, 60]  ParK=[180, 3200, 1]  TcD=1e-4  MaxRateChangeFreq=12  FilterCutOffFreq=25  Ts=0  AGC=on
  PLL (3ph)3 : powerlib_meascontrol/PLL/PLL (3ph)  Commented=on  Fmin=45  Par_Init=[0, 60]  ParK=[180, 3200, 1]  TcD=1e-4  MaxRateChangeFreq=12  FilterCutOffFreq=25  Ts=0  AGC=on
  PLL (3ph)4 : powerlib_meascontrol/PLL/PLL (3ph)  Commented=on  Fmin=45  Par_Init=[0, 60]  ParK=[180, 3200, 1]  TcD=1e-4  MaxRateChangeFreq=12  FilterCutOffFreq=25  Ts=0  AGC=on
  "Power (3ph, Phasor)7" : powerlib_meascontrol/Measurements/Power (3ph, Phasor)  Commented=on
      settings: SourceProductBaseCode=PS
  "Power (3ph, Phasor)8" : powerlib_meascontrol/Measurements/Power (3ph, Phasor)  Commented=on
      settings: SourceProductBaseCode=PS
  "Power (3ph, Phasor)9" : powerlib_meascontrol/Measurements/Power (3ph, Phasor)  Commented=on
      settings: SourceProductBaseCode=PS
  Power Measurement (Three-Phase) : eePowerMeasurement/Power Measurement (Three-Phase)  Commented=on  LabelModeActiveChoice=Continuous  F=60  K=[0 1 2 3]  Seq=Positive  Ts=0
      settings: SourceProductBaseCode=PS
  Power Measurement (Three-Phase){1..3,12..18,21..24,26..30,32..34} (22 alike) : eePowerMeasurement/Power Measurement (Three-Phase)  Commented=on  LabelModeActiveChoice=Discrete  F=60  K=[1]  Seq=Positive  Ts=Ts
      settings: SourceProductBaseCode=PS
  Power Measurement (Three-Phase){4..5,7..10,20} (7 alike) : eePowerMeasurement/Power Measurement (Three-Phase)  LabelModeActiveChoice=Discrete  F=60  K=[1]  Seq=Positive  Ts=Ts
      settings: SourceProductBaseCode=PS
  Power Measurement (Three-Phase){11,19,25,31} (4 alike) : eePowerMeasurement/Power Measurement (Three-Phase)  Commented=on  LabelModeActiveChoice=Discrete  F=60  K=[1]  Seq=Negative  Ts=Ts
      settings: SourceProductBaseCode=PS
  Power Measurement (Three-Phase)6 : eePowerMeasurement/Power Measurement (Three-Phase)  LabelModeActiveChoice=Discrete  F=60  K=[1]  Seq=Negative  Ts=Ts
      settings: SourceProductBaseCode=PS
  RMS : powerlib_meascontrol/Measurements/RMS  Commented=on  TrueRMS=on  Freq=60  RMSInit=120  Ts=0
  RMS2 : powerlib_meascontrol/Measurements/RMS  Commented=on  TrueRMS=on  Freq=60  RMSInit=120  Ts=0
  RMS3 : powerlib_meascontrol/Measurements/RMS  Commented=on  TrueRMS=on  Freq=60  RMSInit=575  Ts=Ts
  Repeating Sequence : simulink/Sources/Repeating Sequence  Commented=on  rep_seq_t=[0 0.1 0.2 0.3 0.4 0.5]  rep_seq_y="1000*[0.7 0.6 0.4 0.8  1 0.7]"
  Repeating Sequence1 : simulink/Sources/Repeating Sequence  Commented=on  rep_seq_t=[0 0.1 0.2 0.3 0.4 0.5]  rep_seq_y="11*[1 1 1 1  1 1]"
  Resource Timeseries : Subsystem
  SL : powerlib/Measurements/Three-Phase V-I Measurement  Commented=on  VoltageMeasurement=phase-to-ground  SetLabelV=on  LabelV=Vabc_SL  Vpu=on  VpuLL=off  CurrentMeasurement=yes  SetLabelI=on  LabelI=Iabc_SL  Ipu=on  Pbase=10e6  Vbase=13200  OutputType=Magnitude  PhasorSimulation=off  PSBequivalent=0
      settings: SourceProductBaseCode=MT,PS
  Scope : Scope  Commented=on  NumInputPorts=5
  Scope{1,5,7,18} (4 alike) : Scope  Commented=on  NumInputPorts=2
  Scope{9..10,13..14} (4 alike) : Scope
  Scope11 : Scope  Commented=on  NumInputPorts=3
  Scope12 : Scope  Commented=on
  Scope15 : Scope  Commented=on
  Scope16 : Scope  Commented=on  NumInputPorts=12
  Scope17 : Scope  Commented=on  NumInputPorts=12
  Scope19 : Scope  Commented=on  NumInputPorts=7
  Scope2 : Scope  NumInputPorts=10
  Scope20 : Scope  Commented=on  NumInputPorts=9
  Scope3 : Scope  Commented=on  NumInputPorts=8
  Scope4 : Scope  Commented=on  NumInputPorts=8
  Scope6 : Scope  Commented=on  NumInputPorts=5
  Scope8 : Scope  NumInputPorts=3
  Sequence Analyzer{,5,14,16..17} (5 alike) : powerlib_meascontrol/Measurements/Sequence Analyzer  Commented=on  Freq=60  n=1  seq=Positive  InInit=[1, 0]  Ts=Ts
      settings: SourceProductBaseCode=PS
  Sequence Analyzer{1..2,6..13} (10 alike) : powerlib_meascontrol/Measurements/Sequence Analyzer  Commented=on  Freq=60  n=1  seq=Negative  InInit=[1, 0]  Ts=Ts
      settings: SourceProductBaseCode=PS
  Sequence Analyzer15 : powerlib_meascontrol/Measurements/Sequence Analyzer  Freq=60  n=1  seq=Positive  InInit=[1, 0]  Ts=Ts
      settings: SourceProductBaseCode=PS
  Sequence Analyzer3 : powerlib_meascontrol/Measurements/Sequence Analyzer  Freq=60  n=1  seq=Positive  InInit=[1, 0]  Ts=Ts
      settings: SourceProductBaseCode=PS
  Sequence Analyzer4 : powerlib_meascontrol/Measurements/Sequence Analyzer  Freq=60  n=1  seq=Positive  InInit=[1, 0]  Ts=Ts
      settings: SourceProductBaseCode=PS
  Signal Editor : SignalEditorBlockLib/Signal Editor  FileName=grid2island_closed_unplanned.mat  ActiveScenario=Transitions  ActiveSignal=Breaker Open Req  IsBus=off  OutputBusObjectStr=Bus: <object name>  SampleTime=0  Interpolate=off  ZeroCross=off  OutputAfterFinalValue=Setting to zero  Unit=inherit  PreserveSignalName=on
  SignalGen : SignalEditorBlockLib/Signal Editor  Commented=on  FileName=breaker_ctlr_isolated.mat  ActiveScenario=QStep222kVAr  ActiveSignal=pstep  IsBus=off  OutputBusObjectStr=Bus: BusObject  SampleTime=0  Interpolate=off  ZeroCross=off  OutputAfterFinalValue=Setting to zero  Unit=inherit  PreserveSignalName=on
  Stab1 : Subsystem  Commented=on
  "Step load. 240 kW in paper " : powerlib/Elements/Three-Phase Parallel RLC Load  LConnTagsString=A|B|C  Configuration=Y (grounded)  NominalVoltage=13200  Vabc=[1e3 1e3 1e3]  Vabcp=[1e3 1e3 1e3]  NominalFrequency=60  UnbalancedPower=off  ActivePower=15e5  InductivePower=0  CapacitivePower=0  Pabc=[10e3 9e3 11e3]  QLabc=[100 90 110]  QCabc=[100 90 110]  Pabcp=[10e3 9e3 11e3]  QLabcp=[100 90 110]  QCabcp=[100 90 110]  Measurements=None  LoadType=constant PQ
      settings: SourceProductBaseCode=MT,PS
  Subsystem1 : Subsystem
  Subsystem2 : Subsystem
  Subsystem4 : Subsystem
  Sum : Sum  Inputs=|++
  Sum1 : Sum  Commented=on  Inputs=-++++++
  Sum2 : Sum  Commented=on  Inputs=-++++
  Sum3 : Sum  Commented=on  Inputs=|++
  Sum4 : Sum  Commented=on  Inputs=|++
  THD : powerlib_meascontrol/Measurements/THD  Freq=60  Ts=0
  Terminator : Terminator
  Terminator1 : Terminator  Commented=on
  Terminator2 : Terminator
  Terminator3 : Terminator  Commented=on
  Terminator4 : Terminator  Commented=on
  Three-Phase Dynamic Load : powerlib/Elements/Three-Phase Dynamic Load  Commented=on  NominalVoltage=[ 13.2e3 60 ]  ActiveReactivePowers=[135e3 32e3]  PositiveSequence=[0.998 -0.0038]  ExternalControl=on  NpNq=[1.3 2]  TimeConstants="[0  0  0  0]"  MinimumVoltage=0.7  Tfilter=1e-2  LoadFlowParameters=[4,0,0,0,0]
      settings: SourceProductBaseCode=PS
  Three-Phase Parallel RLC Load : powerlib/Elements/Three-Phase Parallel RLC Load  LConnTagsString=A|B|C  Configuration=Y (grounded)  NominalVoltage=460  Vabc=[1e3 1e3 1e3]  Vabcp=[1e3 1e3 1e3]  NominalFrequency=60  UnbalancedPower=off  ActivePower=1e3  InductivePower=0  CapacitivePower=0  Pabc=[10e3 9e3 11e3]  QLabc=[100 90 110]  QCabc=[100 90 110]  Pabcp=[10e3 9e3 11e3]  QLabcp=[100 90 110]  QCabcp=[100 90 110]  Measurements=None  LoadType=constant Z
  Three-Phase Transformer (Two Windings)2 : powerlib/Elements/Three-Phase Transformer (Two Windings)  Winding1Connection=Delta (D1)  Winding2Connection=Yg  CoreType=Three single-phase transformers  SetSaturation=off  Hysteresis=off  DataFile='hysteresis'  SetInitialFlux=off  Measurements=None  UNITS=pu  NominalPower=[ 2e6 , 60 ]  Winding1=[13.2e+3 0.006 0.04]  Winding2=[460 0.006 0.04]  Rm=500.02  Lm=500  L0=0.5  Saturation=[0 0;0.0024 1.2;1 1.52]  InitialFluxes=[ 0.8 , -0.8 , 0.7 ]  BreakLoop=off  DiscreteSolver=Trapezoidal iterative  DataType=off  TransfoNumber=1
  Three-Phase Breaker : powerlib/Elements/Three-Phase Breaker  InitialState=closed  SwitchA=on  SwitchB=on  SwitchC=on  SwitchTimes="[1/60  5/60]"  External=on  BreakerResistance=0.01  SnubberResistance=1e6  SnubberCapacitance=inf  Measurements=None
  Three-Phase Breaker1 : powerlib/Elements/Three-Phase Breaker  InitialState=open  SwitchA=on  SwitchB=on  SwitchC=on  SwitchTimes="[1/60  5/60]"  External=on  BreakerResistance=0.01  SnubberResistance=1e6  SnubberCapacitance=inf  Measurements=None
  Three-Phase Breaker2 : powerlib/Elements/Three-Phase Breaker  InitialState=closed  SwitchA=on  SwitchB=on  SwitchC=on  SwitchTimes="[1/50  20/50]"  External=on  BreakerResistance=0.001  SnubberResistance=1e6  SnubberCapacitance=inf  Measurements=None
  Three-Phase Breaker3 : powerlib/Elements/Three-Phase Breaker  InitialState=open  SwitchA=on  SwitchB=on  SwitchC=on  SwitchTimes="[1/60  5/60]"  External=on  BreakerResistance=0.01  SnubberResistance=1e6  SnubberCapacitance=inf  Measurements=None
  Three-Phase Breaker4 : powerlib/Elements/Three-Phase Breaker  InitialState=closed  SwitchA=on  SwitchB=on  SwitchC=on  SwitchTimes="[1/60  5/60]"  External=on  BreakerResistance=0.01  SnubberResistance=1e6  SnubberCapacitance=inf  Measurements=None
  Three-Phase Fault : powerlib/Elements/Three-Phase Fault  InitialStates=0  FaultA=on  FaultB=on  FaultC=on  GroundFault=on  SwitchTimes="[600/60  605/60]"  External=off  SwitchStatus=NaN  FaultResistance=0.001  GroundResistance=0.01  SnubberResistance=1e6  SnubberCapacitance=inf  Measurements=None
  Transformer 1-MVA 13.2-kV/400-V1 : powerlib/Elements/Three-Phase Transformer (Two Windings)  Winding1Connection=Delta (D1)  Winding2Connection=Yg  CoreType=Three single-phase transformers  SetSaturation=off  Hysteresis=off  DataFile='hysteresis'  SetInitialFlux=off  Measurements=None  UNITS=pu  NominalPower=[ 1e6 , 60 ]  Winding1=[13.2e+3 0.002 0.03]  Winding2=[575 0.002 0.03]  Rm=500.02  Lm=500  L0=0.5  Saturation=[0 0;0.0024 1.2;1 1.52]  InitialFluxes=[ 0.8 , -0.8 , 0.7 ]  BreakLoop=off  DiscreteSolver=Trapezoidal iterative  DataType=off  TransfoNumber=1
  Unit Delay : UnitDelay  Commented=on  SampleTime=200e-6  HasFrameUpgradeWarning=on
  Wind Turbine Type 4 : Subsystem  LoadFcn=%find_system(gcs,'FollowLinks', 'on', 'LookUnderMasks', 'all');  mask(Wind Turbine: Model 7){Nb_wt=1, ShowParameters=Converters data for 1 wind turbine, nom=[618460*oversize 730 60], Reactances=[ 1.305, 0.296, 0.252, 0.474,  0.243,  0.18 ], Time_constants=[  4.49  0.0681  0.0513  ], Resistance=0.006, mec=[0.62 0.01 1], init=[ 0  0  0  0  0  0  0  0  1 ], Vnom=575, Imax_grid_conv=1.1, RL_grid=[ 0.15 0.15/50], C_var_filter1=150e3, Vdc_nom=1100, C_DClink1=90000e-6, L_R_Boost=[0.0012     5e-3], Pmec1=618460, wind_speed_CpMax=11.7, wind0=15, DisplayTurbChar=off, H_WT=6.3549, Ksh=0.0446, D_mutual=1.5, w_wt0=1, torque0=1, Kdc=[1.1   27.5]/1, Ki_var_reg=0.05*2.5, Ki_volt_reg=2*2, Kgrid_side_cur_reg=[1  50]*1, Kspeed=[5 1]*2.2, Kboost_cur_reg=[0.025 100], Kp_pitch=15, Kcompensation=[1.5  6], Kfield=[10  20], pitch_max=27, pitch_rate=10, Ts=Ts, FRT_Mode=FRT Mode 1 (I_reactive support), FRT1_triggers=[0.98 1.02 0.0 50], FRT1_k_vrt=[5.4 4.45]*10, FRT2_triggers=[0.6 1.1 0.0 12], FRT2_ramp=[0.5 0.2 0], u_protect=[1.2 0.16 0.0 2], f_protect=[1.1 0.16 0.85 0.16]}
      mask prompts: Nb_wt "Number of wind turbines:"; ShowParameters "Display:"; nom "Nom. power, L-L volt. and freq.: [Pn (VA), Vn (Vrms), fn (Hz)]"; Reactances "Reactances [Xd Xd' Xd'' Xq Xq'' Xl] (p.u.):"; Time_constants "Time constants [Tdo' Tdo'' Tq''] (s):"; Resistance "Resistance Rs (p.u.):"; mec "Inertia constant, friction factor, and pairs of poles: [ H(s)  F(p.u.)  p ]"; init "Initial conditions: [dw(%) th(deg) ia,ib,ic(pu) pha,phb,phc(deg) Vf(pu)]:"; Vnom "Grid-side converter nominal AC voltage (V):"; Imax_grid_conv "Grid-side converter maximum AC current (pu based on generator power and converter nominal AC voltage):"; RL_grid "Grid-side coupling inductor [ L(pu) R(pu),pu based on generator power and converter nominal AC voltage] :"; C_var_filter1 "Line filter capacitor (Q=50) (var):"; Vdc_nom "Nominal DC bus voltage (V)"; C_DClink1 "DC bus capacitor (F):"; L_R_Boost "Boost converter inductance [L(H) R(ohm)]:"; Pmec1 "Nominal mechanical output power (W):"; wind_speed_CpMax "Wind speed at nominal speed and at Cp max (must be between 6 m/s and 30 m/s) (m/s):"; wind0 "Initial wind speed (m/s):"; DisplayTurbChar "Display wind turbine power characteristics:"; H_WT "Wind turbine inertia constant H (s):"; Ksh "Shaft spring constant refer to high-speed shaft (pu of nominal mechanical torque/rad):"; D_mutual "Shaft mutual damping (pu of nominal mechanical torque/pu dw):"; w_wt0 "Turbine initial speed (pu of nominal speed):"; torque0 "Initial output torque (pu of nominal mechanical torque):"; Kdc "DC bus voltage regulator gains [Kp Ki]:"; Ki_var_reg "Grid-side converter var regulator gain [ Ki]:"; Ki_volt_reg "Grid-side converter voltage regulator gain [ Ki]:"; Kgrid_side_cur_reg "Grid-side converter current regulator gains [Kp Ki]:"; Kspeed "Speed regulator gains [Kp Ki]:"; Kboost_cur_reg "Boost inductor current regulator gains [Kp Ki]:"; Kp_pitch "Pitch controller gain [Kp]:"; Kcompensation "Pitch compensation gains [Kp Ki]:"; Kfield "Field excitation gains [Kp Ki]:"; pitch_max "Maximum pitch angle (deg):"; pitch_rate "Maximum rate of change of pitch angle (deg/s)"; Ts "Sample time (s):"; FRT_Mode "Fault-ride-through (FRT) Strategy:"; FRT1_triggers "UVRT-trigger, OVRT-trigger, FRT-band (pu) and FRT-maxTime (s):"; FRT1_k_vrt "Proportional gains [k_UVRT k_OVRT]:"; FRT2_triggers "UVRT-trigger, OVRT-trigger, FRT-band (pu) and FRT-maxTime (s):"; FRT2_ramp "P and Q ramp-up times in (s) and start-delay (s):"; u_protect "Voltage protection [Vmax(pu) Vmax_delay(s) Vmin(pu) Vmin_delay(s)]:"; f_protect "Frequency protection [fmax(pu) fmax_delax(s) fmin(pu) fmin_delay(s)]:"
      mask help: This block implements a model of a variable speed pitch controlled wind turbine using a synchronous generator.
      mask init:
      | %% IEEE 1547
      | OF2 = 62
      | OF1 = 61.2
      | UF1 = 58.5
      | UF2 = 56.5
      | db  = 0.036
      | k   = 0.05
      | 
      | OV2 = 1.2
      | OV1 = 1.1
      | UV1 = 0.88
      | UV2 = 0.5
      | Vdb = 0.02
      | 
      | 
      | %%%%%%%%%%%%%%%%%%%%%%%%%%%%%%%%%%Data porting and initialization for FRT%%%%%%%%%%%%%%% 
      | Nb_WT = Nb_wt;
      | f_rated = nom(3);   % Trying to take from form input
      | U_rated = Vnom; % Check its relation with L-L voltage
      | 
      | %% WEC Parameters:
      | %P_rated = 2e6;
      | %i_rated = sqrt(2)*abs((P_rated-j*(Q_rated))/(sqrt(3)*U_rated));
      | i_rated = 1;
      | i_max = 1.075*i_rated;
      | %f_boost = 2e3;
      | %f_chopper = 2e3;
      | %Vdc_ref = 1250;
      | 
      | %% Extract References:
      | % Measurement Filter (Voltage):
      | f_cut_volt = 10e3; % [Hz]
      | zeta_filt_volt = 1/sqrt(2); % [-]
      | % Measurement Filter (Voltage):
      | f_cut_curr = 10e3; % [Hz]
      | zeta_filt_curr = 1/sqrt(2); % [-]
      | % PLL:
      | pll_Ki = 2.13; % [-]
      | pll_Kp = 0.1775; % [-]
      | 
      | %% FRT:
      | if FRT_Mode == 1
      |     u_uvrt = FRT1_triggers(1);
      |     u_ovrt = FRT1_triggers(2);
      |     frt_band = FRT1_triggers(3);
      |     FRT_maxTime = FRT1_triggers(4);
      |     k_uvrt = max(FRT1_k_vrt(1),0); % limit low to 0
      |     k_uvrt = min(FRT1_k_vrt(1),10); % limit max to 10
      |     k_ovrt = max(FRT1_k_vrt(2),0); % limit low to 0
      |     k_ovrt = min(FRT1_k_vrt(2),10); % limit low to 10
      |     FRT2_ramp_p = 0;
      |     FRT2_ramp_q = 0;
      |     FRT2_delay  = 0;
      | elseif FRT_Mode == 2
      |     u_uvrt = FRT2_triggers(1);
      |     u_ovrt = FRT2_triggers(2);
      |     frt_band = FRT2_triggers(3);
      |     FRT_maxTime = FRT2_triggers(4);
      |     FRT2_ramp_p = FRT2_ramp(1);
      |     FRT2_ramp_q = FRT2_ramp(2);
      |     FRT2_delay  = min(FRT2_ramp(3),1); % limt low to 1s
      |     k_uvrt = 0;
      |     k_ovrt = 0;
      | end
      | 
      | %% Protection settings:
      | umax_protection = u_protect(1);
      | umax_delay = u_protect(2);
      | umin_protection = u_protect(3);
      | umin_delay = u_protect(4);
      | fmax_protection = f_protect(1);
      | fmax_delay = f_protect(2);
      | fmin_protection = f_protect(3);
      | fmin_delay = f_protect(4);
      | 
      | %% Three-phase breaker;
      | Ron_breaker = 1e-9; % [Ohm]
      | Rs_breaker = 1e6; % [Ohm]
      | Cs_breaker = 1e9; % [F]
      | 
      | %% Output Filter:
      | L1_filter = 150e-6; % [H]
      | Rshunt_filter = 0.25; % [Ohm]
      | Lshunt_filter = 15e-3; % [H]
      | Cshunt_filter = 1300e-6; % [F]
      | L2_filter = 5e-6; % [H]
      | 
      | 
      | %%%%%%%%
      | 
      | Vdc_ref=Vdc_nom;   % Here I have set Vdc_ref (=1200) to Vdc_nom = 1100 (Input)
      | % Vdc_ref = 1250;
      | C2_V0 = 0.9*(Vdc_ref); % [V]
      | 
      | % Vdc control:
      | Vdc1_lowLim = 0; % [V]
      | Vdc1_Kp = 0.75; 
      | Vdc1_Ki = 0.075;
      | Vdc1_stateInit = 0.4; 
      | 
      | 
      | % Vdc2 control:
      | Vdc2_tau = 2*inv(f_rated); % [s]
      | Vdc2_filt_init = C2_V0; % [V]
      | Vdc2_Kp = 10; 
      | Vdc2_Ki = 75; 
      | Vdc2_stateInit = 1760; % scaled it to the level of Vdc_nom of 1100
      | %Vdc2_stateInit = 2000; % [V]
      | % Reactive power control:
      | Q_Kp = 1e-3; % proportional gain
      | Q_Ki = 0.035; % integral gain
      | Q_stateInit = 0; % [V]
      | 
      | %%%%%%%%%%%%%%%%%%%%%%%%%%%%%%%%%%%%%%%%%%%%%%%%%%%%%%%%%%%%%%%%%%%%%%%%%%%%%%%%%%%%%%%%%
      | 
      | %Generator data
      | Pnom=nom(1)*Nb_wt;
      | Q_rated = Pnom*0.75;
      | Vnom_gen=nom(2);
      | Fnom=nom(3);
      | Xd=Reactances(1);
      | Xd1=Reactances(2);
      | Xd2=Reactances(3);
      | Xq=Reactances(4);
      | Xq2=Reactances(5);
      | Xl=Reactances(6);
      | Tdo1=Time_constants(1);
      | Tdo2=Time_constants(2);
      | Tq2=Time_constants(3);
      | H=mec(1);
      | F=mec(2);
      | p=mec(3);
      | 
      | % Converters data
      | L_RL=RL_grid(1);
      | R_RL=RL_grid(2);
      | L_Boost=L_R_Boost(1)/Nb_wt;
      | R_Boost=L_R_Boost(2)/Nb_wt;
      | Q_filter=50;
      | C_DClink=C_DClink1*Nb_wt;
      | C_var_filter=C_var_filter1*Nb_wt;
      | 
      | % Controller data
      | Freq_filter=10000;   %Hz
      | Zeta_filter=0.707;
      | Kp_dc=Kdc(1);
      | Ki_dc=Kdc(2);
      | Kp_grid_side_cur_reg=Kgrid_side_cur_reg(1);
      | Ki_grid_side_cur_reg=Kgrid_side_cur_reg(2);
      | Kp_speed=Kspeed(1);
      | Ki_speed=Kspeed(2);
      | Kp_boost_cur_reg=Kboost_cur_reg(1);
      | Ki_boost_cur_reg=Kboost_cur_reg(2);
      | Kp_compensation=Kcompensation(1);
      | Ki_compensation=Kcompensation(2);
      | Kp_field=Kfield(1);
      | Ki_field=Kfield(2);
      | Mod_index_max=1.1;
      | T_speed=5;      %Speed reference time constant (s)
      | Iq_ref_limit_time_constant=0.3; %(s)
      | Current_reg_output_limit=1.1;   %(pu)
      | Var_reg_output_hi_limit=1.1;    %(pu)
      | Var_reg_output_low_limit=0.9;   %(pu)
      | Pitch_time_constant=0.01;       %(s)
      | Vf_limit=10;    %Field voltage limit (pu)
      | Flux_meas_time_constant=1*(1/Fnom); %(s)
      | Ts_snub=50e-6;  %Sample time to compute snubber resistance
      | 
      | 
      | % Turbine data
      | Pmec=Pmec1*Nb_wt;
      | c1 = 0.6450;
      | c2 = 116;
      | c3 = .4;
      | c4 = 5;
      | c5 = 21;
      | c6 = .00912;  % Set Pmin in stall condition (does not vary with wind_speed_Pmax)
      | c7 = .08;
      | c8 = .035;
      | theta=0;
      | CpMax=.465;     %.5;
      | lambda_CpMax=6; %9.9495;
      | 
      | c1_c8=[c1 c2 c3 c4 c5 c6 c7 c8];
      |   
      | 
      | %   Cp = c1*(c6*lambda + (-c4 - c3*(2.5 + theta) + c2*(1/(lambda + ...
      | %   c7*(2.5 + theta)) - c8/(1 + (2.5 + theta)^3)))/exp(c5*(1/(lambda + ...
      | %   c7*(2.5 + theta)) - c8/(1 + (2.5 + theta)^3))))
      | 
      | 
      |         %%%%%%%%%%%%%%%%%%%%%%%%%%%%%%%%%%%%%%%%%%%%%%%%%%%%%%%%%%%%%%%%%%%%%%%%%%%
      |         % Operation at Cp max
      |         %%%%%%%%%%%%%%%%%%%%%%%%%%%%%%%%%%%%%%%%%%%%%%%%%%%%%%%%%%%%%%%%%%%%%%%%%%%
      |         
      |         rated_omegar=1;
      |         omegar = rated_omegar;
      |         
      |         % Enforce boundaries on wind speed
      |         % A warning could be displayed
      |         if wind_speed_CpMax < 6
      |             wind_speed_CpMax=6;
      |             disp('Warning: Wind speed at nominal speed and at Cp max has been set to 6 m/s')
      |         end
      |         if wind_speed_CpMax > 30
      |             wind_speed_CpMax=30;
      |             disp('Warning: Wind speed at nominal speed and at Cp max has been set to 30 m/s')
      |         end
      | 
      |         K1=lambda_CpMax/omegar*wind_speed_CpMax;
      |         
      |         % Calculation of K2 needed to get P equal to the requested value at
      |         % Cp max for the requested wind speed
      |         
      |         Prated=Pmec;
      |         P_rated_omegar_theta_zero=1; %0.75;
      |         
      |         K2 = P_rated_omegar_theta_zero*Prated/(wind_speed_CpMax^3*CpMax);
      |         
      |         K1_K2=[K1 K2];
      |         
      |         %%%%%%%%%%%%%%%%%%%%%%%%%%%%%%%%%%%%%%%%%%%%%%%%%%%%%%%%%%%%%%%%%%%%%%%%%%%
      |         % End of calculation for operation at Cp max
      |         %%%%%%%%%%%%%%%%%%%%%%%%%%%%%%%%%%%%%%%%%%%%%%%%%%%%%%%%%%%%%%%%%%%%%%%%%%%
      |         
      | 
      | %%%%%%%%%%%%%%%%%%%%%%%%%%%%%%%%%%%%%%%%%%%%%%%%%%%%%%%%%%%%%%%%%%%%%%%%%%%
      | % Plot turbine characteristics
      | %%%%%%%%%%%%%%%%%%%%%%%%%%%%%%%%%%%%%%%%%%%%%%%%%%%%%%%%%%%%%%%%%%%%%%%%%%% 
      | 
      | DisplayTurbChar=get_param(gcb,'DisplayTurbChar');
      | if strcmp(DisplayTurbChar,'on')
      |     vect_theta = 0:2:30;
      |     
      |     vect_lambda = 1:0.2:30;
      |     
      |     clear Cp;
      |     
      |     for i=1:length(vect_theta)
      |      for j=1:length(vect_lambda)
      |                 Cp(i,j) = c1*(c6*vect_lambda(j) + (-c4 - c3*(2.5 + vect_theta(i)) + c2*(1/(vect_lambda(j) + ...
      |                 c7*(2.5 + vect_theta(i))) - c8/(1 + (2.5 + vect_theta(i))^3)))/exp(c5*(1/(vect_lambda(j) + ...
      |                 c7*(2.5 + vect_theta(i))) - c8/(1 + (2.5 + vect_theta(i))^3))));
      |      end
      |     end
      | 
      |     figure(1);
      |     clf;
      |     hold on;
      | 
      |     plot(vect_lambda, Cp);
      |     axis([0, 25, 0, .6]);
      |     title('Wind Turbine Cp Characteristic (pitch angle increases by step of 2 deg.)');
      |     ylabel('Cp');
      |     set(gca,'ytick',[0 .1 .2 .3 .4 .5 .6]);
      |     xlabel('Lambda');
      |     grid on;
      |     text(10.1,0.51,'Pitch angle 0 degree');
      | 
      |     hold off
      |     
      |     % Plot of the wind turbine mechanical power output (pu) lambda and Cp
      |     % characteristics against wind speed (m/s) for a range of theta.
      |     
      |     wind_speed_range = [1,.2,30];
      |     vect_wind_speed = 1:0.2:30;
      |     
      |     clear lambda;
      |     clear Cp;
      |     clear P;
      | 
      |     for i=1:length(vect_theta)
      |         for j=1:length(vect_wind_speed)
      |             lambda(i,j) = K1*omegar/vect_wind_speed(j);
      |             Cp(i,j) = c1*(c6*lambda(i,j) + (-c4 - c3*(2.5 + vect_theta(i)) + c2*(1/(lambda(i,j) + ...
      |             c7*(2.5 + vect_theta(i))) - c8/(1 + (2.5 + vect_theta(i))^3)))/exp(c5*(1/(lambda(i,j) + ...
      |             c7*(2.5 + vect_theta(i))) - c8/(1 + (2.5 + vect_theta(i))^3))));
      |             P(i,j) = K2/Prated*vect_wind_speed(j)^3*Cp(i,j);
      |         end
      |     end
      |     
      |     
      |     figure(2);
      |     clf;
      |     hold on
      |     
      |     subplot(3,1,1);
      |     plot(vect_wind_speed, P);
      |     axis([0, 35, 0, 1.5]);
      |     title('Wind Turbine Characteristics (w = 1 pu, pitch angle increases by step of 2 deg.)');
      |     ylabel('P (pu)');
      |     set(gca,'ytick',0:.5:4);
      |     grid on;
      |     
      |     subplot(3,1,2);
      |     plot(vect_wind_speed, lambda);
      |     axis([0, 35, 0, 20]);
      |     ylabel('Lambda');
      |     grid on;
      |     
      |     subplot(3,1,3)
      |     plot(vect_wind_speed, Cp);
      |     axis([0, 35, 0, .6]);
      |     xlabel('Wind Speed (m/s)');
      |     ylabel('Cp');
      |     set(gca,'ytick',[0 .1 .2 .3 .4 .5 .6]);
      |     grid on;
      | 
      |     hold off
      |     set_param(gcb,'DisplayTurbChar','off')
      |     
      | end
      mask TypeOptions ShowParameters: Generator data for 1 wind turbine | Converters data for 1 wind turbine | Turbine data for 1 wind turbine | Drive train data for 1 wind turbine | Control parameters for 1 wind turbine | Fault-ride-through (FRT) Strategy
      mask Callback ShowParameters:
      | BlockName=getfullname(gcb);
      | %
      | Param_Show=get_param(BlockName,'ShowParameters');
      | Param_DisplayTurbChar=get_param(BlockName,'DisplayTurbChar');
      | 
      | p_mask{3}='off';p_mask{4}='off';p_mask{5}='off';
      | p_mask{6}='off';p_mask{7}='off';p_mask{8}='off';p_mask{9}='off';
      | p_mask{10}='off';p_mask{11}='off';p_mask{12}='off';p_mask{13}='off';
      | p_mask{14}='off';p_mask{15}='off';p_mask{16}='off';p_mask{17}='off';
      | p_mask{18}='off';p_mask{19}='off';p_mask{20}='off';p_mask{21}='off';
      | p_mask{22}='off';p_mask{23}='off';p_mask{24}='off';p_mask{25}='off';
      | p_mask{26}='off';p_mask{27}='off';p_mask{28}='off';p_mask{29}='off';
      | p_mask{30}='off';p_mask{31}='off';p_mask{32}='off';p_mask{33}='off';
      | p_mask{34}='off';p_mask{35}='off';
      | p_mask{37}='off';p_mask{38}='off';p_mask{39}='off';p_mask{40}='off';
      | p_mask{41}='off';p_mask{42}='off';p_mask{43}='off';
      | 
      | switch Param_Show
      | 	case 'Generator data for 1 wind turbine'
      | 		p_mask{3}='on';p_mask{4}='on';p_mask{5}='on';
      |         p_mask{6}='on';p_mask{7}='on';p_mask{8}='on';
      |     case 'Converters data for 1 wind turbine'
      | 		p_mask{9}='on';p_mask{10}='on';p_mask{11}='on';
      |         p_mask{12}='on';p_mask{13}='on';p_mask{14}='on';p_mask{15}='on';
      | 	case 'Turbine data for 1 wind turbine'
      | 		p_mask{16}='on';p_mask{17}='on';p_mask{18}='on';p_mask{19}='on';
      |     case 'Drive train data for 1 wind turbine'
      |         p_mask{20}='on';p_mask{21}='on';p_mask{22}='on';p_mask{23}='on';
      |         p_mask{24}='on';
      |     case 'Control parameters for 1 wind turbine'
      |         p_mask{25}='on';p_mask{26}='on';p_mask{27}='on';
      |         p_mask{28}='on';p_mask{29}='on';p_mask{30}='on';p_mask{31}='on';
      |         p_mask{32}='on';p_mask{33}='on';p_mask{34}='on';p_mask{35}='on';
      |     case 'Fault-ride-through (FRT) Strategy'
      |         p_mask{37}='on';
      |         switch Param_Show
      |         case 'FRT Mode 1 (I_reactive support)'
      |             p_mask{38}='on';p_mask{39}='on';
      |             p_mask{42}='on';p_mask{43}='on';
      |         case 'FRT Mode 2 (Zero power mode)'
      |             p_mask{40}='on';p_mask{41}='on';
      |             p_mask{42}='on';p_mask{43}='on';
      |         end
      | end
      | 
      | ParVisible={'on','on',p_mask{3},p_mask{4},p_mask{5},p_mask{6},...
      |     p_mask{7},p_mask{8},p_mask{9},p_mask{10},p_mask{11},p_mask{12},...
      |     p_mask{13},p_mask{14},p_mask{15},p_mask{16},p_mask{17},p_mask{18},...
      |     p_mask{19},p_mask{20},p_mask{21},p_mask{22},p_mask{23},p_mask{24},...
      |     p_mask{25},p_mask{26},p_mask{27},p_mask{28},p_mask{29},p_mask{30},...
      |     p_mask{31},p_mask{32},p_mask{33},p_mask{34},p_mask{35},'on',...
      |     p_mask{37},p_mask{38},p_mask{39},p_mask{40},p_mask{41},...
      |     p_mask{42},p_mask{43}};
      | %
      | set_param(BlockName,'MaskVisibilities',ParVisible);
      | set_param(BlockName,'DisplayTurbChar',Param_DisplayTurbChar);
      mask TypeOptions FRT_Mode: FRT Mode 1 (I_reactive support) | FRT Mode 2 (Zero power mode)
      mask Callback FRT_Mode:
      | BlockName=getfullname(gcb);
      | 
      | Param_Show=get_param(BlockName,'FRT_Mode');
      | Param_Visible=get_param(BlockName,'MaskVisibilities');
      | Param_Visible{37}='on';
      | Param_Visible{38}='off';Param_Visible{39}='off';Param_Visible{40}='off';Param_Visible{41}='off';
      | Param_Visible{42}='on';Param_Visible{43}='on';
      | switch Param_Show
      | 	case 'FRT Mode 1 (I_reactive support)'
      | 		Param_Visible{38}='on';Param_Visible{39}='on';
      |     case 'FRT Mode 2 (Zero power mode)'
      | 		Param_Visible{40}='on';Param_Visible{41}='on';
      | end
      | 
      | set_param(BlockName,'MaskVisibilities',Param_Visible);
      mask Display: disp(' ');
  Zero-Order Hold : ZeroOrderHold  Commented=on  SampleTime=Ts
  induction attempts2 : Subsystem  Commented=on
      mask Display: image('$imagefile'); % Use "Edit Image" on toolstrip to change.
  powergui : powerlib/powergui  Priority=1  SimulationMode=Discrete  SampleTime=Ts_Power  frequency=60  Iterations=50  frequencyindice=60  Pbase=10e6  ErrMax=0.0001  UnitsV=kV  UnitsW=MW  buscounter=0  FunctionMessages=off  echomessages=off  EnableUseOfTLC=off  CurrentSourceSwitches=off  DisableSnubberDevices=off  DisableRonSwitches=off  DisableVfSwitches=off  DisplayEquations=off  AutomaticDiscreteSolvers=off  SolverType=Tustin/Backward Euler (TBE)  Interpol=off  ExternalGateDelay=off  methode=off  Ts=100  x0status=steady  SPID=on  SwTol=0  HookPort=off  NonlinearTolerance=1e-4  nMaxIteration=100  ContinueOnMaxIteration=off  RestoreLinks=warning  ResistiveCurrentMeasurement=off  Frange=[0:2:500]  Ylog=off  Xlog=on  ShowGrid=off  save=off  variable=ZData  structure=0  ZoomFFT=off  StartTime=0.0  cycles=1  DisplayStyle=1  fundamental=60  FreqAxis=off  MaxFrequency=1000  frequencyindicesteady=1  RmsSteady=2  display=off
  synchronous : Subsystem
      mask Display: image('$imagefile'); % Use "Edit Image" on toolstrip to change.
  uhhh : Subsystem  Commented=on
      mask Display: image('$imagefile'); % Use "Edit Image" on toolstrip to change.
  tag scope: Scenario=global
  wires:
  Mux/1 -> Three-Phase Dynamic Load/1
  Three-Phase Dynamic Load/1 -> Bus Selector3/1
  Bus Selector3/2 -> Active Load/2  "<Reactive power Q (var)>"
  Bus Selector3/1 -> Active Load/1  "<Positive-sequence voltage V (pu)>"
  Bus Selector3/3 -> Active Load/3  "<Active power P (W)>"
  Gain/1 -> Mux/1
  Gain1/1 -> Mux/2
  [Vabc_B1] -> Scope4/1, THD/1  "V_BUS"
  From18/1 -> Scope4/2  "I_GRID"
  From19/1 -> Scope4/3  "I_WIND"
  From20/1 -> Scope4/4  "I_PV"
  From21/1 -> Scope4/5  "I_GEN"
  From22/1 -> Scope4/6  "I_BESS"
  FC_BESS/1(m) -> Bus Selector/1
  Bus Selector/1 -> Scope8/1  "<SOC (%)>"
  Bus Selector/3 -> Scope8/3  "<Voltage (V)>"
  Bus Selector/2 -> Scope8/2  "<Current (A)>"
  Microgrid controller/1(BESS_Control) -> FC_BESS/1(Control)
  FC_PV_FirstSolar/1(m) -> Terminator/1
  Control1/1(Out1) -> FC_PV_FirstSolar/1(Control)
  [SR_ts_wm2] -> FC_PV_FirstSolar/2(Irradiance)
  [Vabc_B1] -> Grid Feeder Protective Relay/2(V_line)
  [Vabc_B2] -> Grid Feeder Protective Relay/3(V_bus)
  [Iabc_B1] -> Grid Feeder Protective Relay/4(I)
  Grid Feeder Protective Relay/1(Meas) -> Microgrid controller/1(ProtRelayMeas), [ProtRelayMeas]
  From9/1 -> Bus Selector1/1
  Bus Selector1/1 -> Scope/1  "<dWt>"
  Bus Selector1/2 -> Scope/2  "<dF>"
  Bus Selector1/3 -> Scope/3  "<dV>"
  Bus Selector1/4 -> Scope/4  "<R25_SyncOK>"
  Bus Selector1/5 -> Scope/5  "<Closed>"
  [Scenario] -> Grid Feeder Protective Relay/1(Ctrl)
  Power Measurement (Three-Phase)8/1 -> Mux2/1  "P(BESS)"
  From29/1 -> Scope3/7  "Vabc_B5"
  From28/1 -> Mux1/1
  From23/1 -> Scope3/5  "Vdc (V)"
  From25/1 -> Scope3/1  "Vabc_B3"
  Demux/1 -> Scope3/3  "P (MW)"
  Demux/2 -> Scope3/4  "Q (Mvar)"
  From17/1 -> Scope3/8  "Iabc_B5"
  MW/1 -> Demux/1
  From26/1 -> Scope3/2  "Iabc_B3"
  From27/1 -> Mux1/2
  Mux1/1 -> MW/1
  From24/1 -> Scope3/6  "wr (pu)"
  Power Measurement (Three-Phase)/2 -> RMS2/1
  RMS2/1 -> Scope5/2
  Power Measurement (Three-Phase)/1 -> RMS/1
  From32/1 -> Power Measurement (Three-Phase)/1
  From33/1 -> Power Measurement (Three-Phase)/2
  RMS/1 -> Scope5/1
  [Scenario] -> Grid Feeder Protective Relay1/1(Ctrl)
  [Iabc_B7] -> Grid Feeder Protective Relay1/4(I)
  [Vabc_B8] -> Grid Feeder Protective Relay1/3(V_bus)
  [Vabc_B7] -> Grid Feeder Protective Relay1/2(V_line)
  Grid Feeder Protective Relay1/1(Meas) -> [GenRelayMeas]
  From42/1 -> Scope4/7  "fcgi"
  THD/1 -> [THD_B1]
  From43/1 -> Scope4/8  "thd"
  Grid Feeder Protective Relay1/2(BreakerClose) -> Three-Phase Breaker2/1, Scope9/1
  From34/1 -> Bus Selector4/1
  Bus Selector4/1 -> Scope6/1  "<dWt>"
  Bus Selector4/2 -> Scope6/2  "<dF>"
  Bus Selector4/3 -> Scope6/3  "<dV>"
  Bus Selector4/4 -> Scope6/4  "<R25_SyncOK>"
  Bus Selector4/5 -> Scope6/5  "<Closed>"
  [Iabc_B7] -> Power Measurement (Three-Phase)5/2
  Power Measurement (Three-Phase)5/1 -> Mux5/1  "P(Gen)"
  [Vabc_B7] -> Power Measurement (Three-Phase)5/1
  Mux2/1 -> Scope2/4  "PQ_BESS"
  Power Measurement (Three-Phase)7/1 -> Mux3/1  "P(PV)"
  Power Measurement (Three-Phase)5/2 -> Mux5/2  "Q(Gen)"
  Power Measurement (Three-Phase)4/1 -> Gain4/1  "P(Grid)"
  [Iabc_B1] -> Power Measurement (Three-Phase)4/2
  [Vabc_B1] -> Power Measurement (Three-Phase)4/1
  Mux3/1 -> Scope2/5  "PQ_PV"
  Power Measurement (Three-Phase)6/1 -> Mux4/1  "P(Wind)"
  Mux4/1 -> Gain10/1  "PQ_Wind"
  [Vabc_B4] -> Power Measurement (Three-Phase)7/1
  Power Measurement (Three-Phase)6/2 -> Mux4/2  "Q(Wind)"
  [Vabc_B3] -> Power Measurement (Three-Phase)6/1
  Power Measurement (Three-Phase)4/2 -> Gain18/1  "Q(Grid)"
  [Iabc_B9] -> Power Measurement (Three-Phase)8/2
  Mux5/1 -> Scope2/7  "PQ_Gen"
  Power Measurement (Three-Phase)7/2 -> Mux3/2  "Q(PV)"
  [Iabc_B3] -> Power Measurement (Three-Phase)6/2
  [Iabc_B4] -> Power Measurement (Three-Phase)7/2
  Power Measurement (Three-Phase)8/2 -> Mux2/2  "Q(BESS)"
  ? -> Goto10/1
  SignalGen/1 -> Goto9/1
  From5/1 -> Zero-Order Hold/1
  Discrete Frequency Regulator/1(Control) -> Unit Delay/1
  Zero-Order Hold/1 -> Discrete Frequency Regulator/1(Vabc)
  Unit Delay/1 -> Defferable Load (0-446.25 kW)/1(Control)
  From48/1 -> Scope7/1  "Vabc_B3"
  From49/1 -> Scope7/2  "Iabc_B3"
  Constant4/1 -> ../1("Wind (m/s) ")
  Bus Selector5/3 -> Goto11/1  "<P_pu>"
  Bus Selector5/4 -> Goto14/1  "<Q_pu>"
  Bus Selector5/1 -> Goto12/1  "<Vdc_V>"
  ../1(m) -> Bus Selector5/1
  Bus Selector5/2 -> Goto13/1  "<wr_pu>"
  PLL (3ph)2/1 -> Scope1/1, Goto19/1  "Freqv3"
  PLL (3ph)2/2 -> Terminator3/1
  From1/1 -> PLL (3ph)2/1
  From50/1 -> RMS3/1
  RMS3/1 -> Demux1/1
  Demux1/1 -> Add/1
  Demux1/2 -> Add/2
  Demux1/3 -> Add/3
  Add/1 -> Gain2/1
  Gain2/1 -> Scope1/2, Goto20/1  "rmsv3"
  Constant/1 -> Gain/1
  Constant7/1 -> Gain1/1
  Constant2/1 -> ../2(Qref_pu)
  Grid Feeder Protective Relay/2(BreakerClose) -> Three-Phase Breaker/1, Scope10/1
  Signal Editor/1 -> Bus Creator/1
  ? -> Bus Creator/7  "BESS_GFM_Ena"
  ? -> Bus Creator/2  "ReqOpen"
  ? -> Bus Creator/4  "ReqClose"
  ? -> Bus Creator/3  "GenReqOpen"
  Bus Creator/1 -> [Scenario]
  ? -> Bus Creator/5  "GenReqClose"
  ? -> Bus Creator/6  "StartResync"
  From Spreadsheet/1 -> Wind Turbine Type 4/2(AS mode)
  Bus Selector2/4 -> [Q_pu]  "<Q_pu>"
  Constant1/1 -> Wind Turbine Type 4/1("Wind (m/s) ")
  Bus Selector2/2 -> [wr]  "<wr_pu>"
  Bus Selector2/1 -> [Vdc]  "<Vdc_V>"
  Bus Selector2/3 -> [P_pu]  "<P_pu>"
  Wind Turbine Type 4/1(m) -> Bus Selector2/1
  Mux6/1 -> Scope2/8  "PQ_grid"
  From40/1 -> Sequence Analyzer/1
  Sequence Analyzer/1 -> Gain6/1  "V_BUS"
  Gain6/1 -> Mux10/1  "V_B1 [pu]"
  From51/1 -> Sequence Analyzer1/1
  Sequence Analyzer1/1 -> Gain8/1  "V_BUS"
  Gain8/1 -> Mux10/2  "V_B2 [pu]"
  Sequence Analyzer2/1 -> Gain11/1  "V_BUS"
  From52/1 -> Sequence Analyzer2/1
  Gain11/1 -> Mux10/3  "V_B3 [pu]"
  Mux10/1 -> Scope12/1  "VB1-12"
  [Vabc_B9] -> Power Measurement (Three-Phase)8/1
  Gain9/1 -> Scope2/2  "V [pu]"
  Sequence Analyzer3/1 -> Gain9/1
  Subsystem1/1(control) -> Scope13/1, Three-Phase Breaker1/1
  [f_B14] -> Subsystem1/1(freq)
  Subsystem2/1(control) -> Scope14/1, Three-Phase Breaker3/1
  Gain10/1 -> Scope2/6  "PQ_wind"
  [Vabc_B14] -> Power Measurement (Three-Phase)9/1
  [Iabc_B14] -> Power Measurement (Three-Phase)9/2
  Power Measurement (Three-Phase)9/1 -> Sum/1  "P(Grid)"
  [Iabc_B15] -> Power Measurement (Three-Phase)10/2
  [Vabc_B15] -> Power Measurement (Three-Phase)10/1
  Power Measurement (Three-Phase)10/1 -> Sum/2  "P(Grid)"
  Sequence Analyzer5/1 -> Gain15/1  "V_BUS"
  Gain15/1 -> Mux10/4  "V_B4 [pu]"
  From60/1 -> Sequence Analyzer5/1
  Sequence Analyzer6/1 -> Gain17/1  "V_BUS"
  From61/1 -> Sequence Analyzer6/1
  Gain17/1 -> Mux10/5  "V_B5 [pu]"
  From62/1 -> Sequence Analyzer7/1
  Sequence Analyzer7/1 -> Gain19/1  "V_BUS"
  Gain19/1 -> Mux10/6  "V_B6 [pu]"
  Sequence Analyzer8/1 -> Gain21/1  "V_BUS"
  From63/1 -> Sequence Analyzer8/1
  Sequence Analyzer9/1 -> Gain23/1  "V_BUS"
  From64/1 -> Sequence Analyzer9/1
  Sequence Analyzer10/1 -> Gain25/1  "V_BUS"
  From65/1 -> Sequence Analyzer10/1
  Sequence Analyzer11/1 -> Gain27/1  "V_BUS"
  From66/1 -> Sequence Analyzer11/1
  Sequence Analyzer12/1 -> Gain29/1  "V_BUS"
  From67/1 -> Sequence Analyzer12/1
  Sequence Analyzer13/1 -> Gain31/1  "V_BUS"
  From68/1 -> Sequence Analyzer13/1
  Gain21/1 -> Mux10/7  "V_B7 [pu]"
  Gain23/1 -> Mux10/8  "V_B8 [pu]"
  Gain25/1 -> Mux10/9  "V_B9 [pu]"
  Gain27/1 -> Mux10/10  "V_B10 [pu]"
  Gain29/1 -> Mux10/11  "V_B11 [pu]"
  Gain31/1 -> Mux10/12  "V_B12 [pu]"
  From69/1 -> "Power (3ph, Phasor)7"/1
  Gain5/1 -> Scope11/1  "PQ_grid"
  "Power (3ph, Phasor)7"/1 -> Mux7/1  "P(Grid)"
  "Power (3ph, Phasor)7"/2 -> Mux7/2  "Q(Grid)"
  Mux7/1 -> Gain5/1
  From70/1 -> "Power (3ph, Phasor)7"/2
  From71/1 -> "Power (3ph, Phasor)8"/1
  Gain7/1 -> Scope11/2  "PQ_grid"
  "Power (3ph, Phasor)8"/1 -> Mux8/1  "P(Grid)"
  "Power (3ph, Phasor)8"/2 -> Mux8/2  "Q(Grid)"
  Mux8/1 -> Gain7/1
  From72/1 -> "Power (3ph, Phasor)8"/2
  Gain12/1 -> Scope11/3  "PQ_grid"
  "Power (3ph, Phasor)9"/2 -> Mux9/2  "Q(Grid)"
  From74/1 -> "Power (3ph, Phasor)9"/2
  "Power (3ph, Phasor)9"/1 -> Mux9/1  "P(Grid)"
  Mux9/1 -> Gain12/1
  From73/1 -> "Power (3ph, Phasor)9"/1
  Gain14/1 -> Scope15/1  "V_B1 [pu]"
  From75/1 -> Sequence Analyzer14/1
  Sequence Analyzer14/1 -> Gain14/1  "V_BUS"
  [Vabc_B13] -> Sequence Analyzer3/1, PLL (3ph)1/1
  PLL (3ph)1/2 -> Terminator2/1
  PLL (3ph)1/1 -> Scope2/1
  Sum/1 -> Gain3/1
  Gain4/1 -> Mux6/1  "P(grid)"
  Gain18/1 -> Mux6/2  "Q(grid)"
  Gain3/1 -> Scope2/9  "PQ_load"
  Constant3/1 -> Three-Phase Breaker4/1
  Bus Selector2/5 -> [Vwtg]  "<Vabc_grid_pu>"
  [Vwtg] -> Sequence Analyzer4/1
  Sequence Analyzer4/1 -> Scope2/10  "V_BUS"
  From81/1 -> Power Measurement (Three-Phase)11/2
  From82/1 -> Power Measurement (Three-Phase)3/1
  From76/1 -> Power Measurement (Three-Phase)12/1
  From83/1 -> Power Measurement (Three-Phase)3/2
  From55/1 -> Power Measurement (Three-Phase)13/2
  From80/1 -> Power Measurement (Three-Phase)11/1
  From91/1 -> Power Measurement (Three-Phase)13/1
  From84/1 -> Power Measurement (Three-Phase)2/1
  From85/1 -> Power Measurement (Three-Phase)2/2
  From87/1 -> Power Measurement (Three-Phase)14/1
  From77/1 -> Power Measurement (Three-Phase)12/2
  From88/1 -> Power Measurement (Three-Phase)14/2
  From89/1 -> Power Measurement (Three-Phase)1/1
  From90/1 -> Power Measurement (Three-Phase)1/2
  From92/1 -> Power Measurement (Three-Phase)15/2
  From86/1 -> Power Measurement (Three-Phase)15/1
  From93/1 -> Power Measurement (Three-Phase)16/1
  From94/1 -> Power Measurement (Three-Phase)16/2
  From96/1 -> Power Measurement (Three-Phase)17/2
  From95/1 -> Power Measurement (Three-Phase)17/1
  From98/1 -> Power Measurement (Three-Phase)18/2
  From97/1 -> Power Measurement (Three-Phase)18/1
  From99/1 -> Power Measurement (Three-Phase)19/1
  From100/1 -> Power Measurement (Three-Phase)19/2
  Power Measurement (Three-Phase)2/1 -> Sum1/1, Scope16/1  "Pgrid"
  Power Measurement (Three-Phase)11/1 -> Scope16/2  "P3"
  Power Measurement (Three-Phase)12/1 -> Sum1/4, Scope16/3  "Psolar"
  Power Measurement (Three-Phase)19/1 -> Sum1/3, Scope16/4  "P5"
  Power Measurement (Three-Phase)3/1 -> Scope16/5  "P7"
  Power Measurement (Three-Phase)18/1 -> Sum1/2, Scope16/6  "P8"
  Power Measurement (Three-Phase)13/1 -> Scope16/7, Sum1/5  "P9"
  Power Measurement (Three-Phase)14/1 -> Scope16/8  "P10"
  Power Measurement (Three-Phase)1/1 -> Scope16/9  "P11"
  Power Measurement (Three-Phase)17/1 -> Scope16/10  "P13"
  Power Measurement (Three-Phase)15/1 -> Sum1/7, Scope16/11  "P14"
  Power Measurement (Three-Phase)16/1 -> Sum1/6, Scope16/12  "P15"
  Power Measurement (Three-Phase)2/2 -> Sum2/1, Scope17/1  "Q1"
  Power Measurement (Three-Phase)11/2 -> Scope17/2  "Q3"
  Power Measurement (Three-Phase)12/2 -> Sum2/4, Scope17/3  "Q4"
  Power Measurement (Three-Phase)19/2 -> Sum2/2, Scope17/4  "Q5"
  Power Measurement (Three-Phase)3/2 -> Scope17/5  "Q7"
  Power Measurement (Three-Phase)18/2 -> Scope17/6, Sum2/3  "Q8"
  Power Measurement (Three-Phase)13/2 -> Scope17/7, Sum2/5  "Q9"
  Power Measurement (Three-Phase)14/2 -> Scope17/8  "Q10"
  Power Measurement (Three-Phase)1/2 -> Scope17/9  "Q11"
  Power Measurement (Three-Phase)17/2 -> Scope17/10  "Q13"
  Power Measurement (Three-Phase)15/2 -> Scope17/11  "Q14"
  Power Measurement (Three-Phase)16/2 -> Scope17/12  "Q14"
  Sum1/1 -> Scope18/1
  Sum2/1 -> Scope18/2
  PLL (3ph)/1 -> [f_B14]  "f"
  [Vabc_B14] -> Sequence Analyzer15/1, PLL (3ph)/1
  [Iabc_B16] -> Power Measurement (Three-Phase)20/2
  Power Measurement (Three-Phase)20/1 -> Mux11/1  "P(BESS)"
  Mux11/1 -> Scope2/3  "PQ_stab"
  [Vabc_B16] -> Power Measurement (Three-Phase)20/1
  Power Measurement (Three-Phase)20/2 -> Mux11/2  "Q(BESS)"
  Control3/1(Control) -> MODEL STABILIZER/1(Control)
  Sequence Analyzer15/1 -> [V_B14]  "V"
  [V_B14] -> Subsystem1/2(Voltage)
  [f_B14] -> Subsystem2/1(freq)
  [V_B14] -> Subsystem2/2(Voltage)
  Power Measurement (Three-Phase)26/1 -> Mux14/1  "P(PV)"
  From118/1 -> Power Measurement (Three-Phase)28/1
  Sequence Analyzer16/1 -> Gain24/1
  From114/1 -> Power Measurement (Three-Phase)24/2
  Mux14/1 -> Scope19/3
  Power Measurement (Three-Phase)25/1 -> Mux15/1  "P(Wind)"
  Power Measurement (Three-Phase)23/1 -> Gain22/1  "P(Grid)"
  From115/1 -> Power Measurement (Three-Phase)23/1
  Power Measurement (Three-Phase)24/1 -> Mux16/1  "P(Gen)"
  Power Measurement (Three-Phase)23/2 -> Gain16/1  "Q(Grid)"
  Power Measurement (Three-Phase)25/2 -> Mux15/2  "Q(Wind)"
  PLL (3ph)3/2 -> Terminator1/1
  Sum3/1 -> Gain20/1
  From112/1 -> Sequence Analyzer16/1, PLL (3ph)3/1
  Mux15/1 -> Gain13/1  "PQ_Wind"
  From108/1 -> Power Measurement (Three-Phase)26/1
  Gain16/1 -> Mux17/2  "Q(grid)"
  Mux16/1 -> Scope19/5
  Power Measurement (Three-Phase)24/2 -> Mux16/2  "Q(Gen)"
  PLL (3ph)3/1 -> Scope19/1
  From111/1 -> Power Measurement (Three-Phase)25/2
  Gain22/1 -> Mux17/1  "P(grid)"
  From109/1 -> Power Measurement (Three-Phase)26/2
  From110/1 -> Power Measurement (Three-Phase)25/1
  From120/1 -> Power Measurement (Three-Phase)21/1
  Power Measurement (Three-Phase)21/1 -> Sum3/2  "crit load"
  Power Measurement (Three-Phase)26/2 -> Mux14/2  "Q(PV)"
  From121/1 -> Power Measurement (Three-Phase)21/2
  From113/1 -> Power Measurement (Three-Phase)24/1
  Gain13/1 -> Scope19/4
  Mux17/1 -> Scope19/6
  From119/1 -> Power Measurement (Three-Phase)28/2
  Power Measurement (Three-Phase)28/1 -> Sum3/1  "deferable load"
  Gain20/1 -> Scope19/7
  From116/1 -> Power Measurement (Three-Phase)23/2
  Gain24/1 -> Scope19/2
  Power Measurement (Three-Phase)27/1 -> Mux12/1  "P(stab)"
  From106/1 -> Power Measurement (Three-Phase)27/1
  Power Measurement (Three-Phase)32/1 -> Mux18/1  "P(PV)"
  Power Measurement (Three-Phase)27/2 -> Mux12/2  "Q(stab)"
  From105/1 -> Power Measurement (Three-Phase)27/2
  From131/1 -> Power Measurement (Three-Phase)34/1
  Sequence Analyzer17/1 -> Gain33/1
  From127/1 -> Power Measurement (Three-Phase)30/2
  Power Measurement (Three-Phase)31/1 -> Mux19/1  "P(Wind)"
  Power Measurement (Three-Phase)29/1 -> Gain32/1  "P(Grid)"
  From128/1 -> Power Measurement (Three-Phase)29/1
  Power Measurement (Three-Phase)30/1 -> Mux20/1  "P(Gen)"
  Power Measurement (Three-Phase)29/2 -> Gain28/1  "Q(Grid)"
  Power Measurement (Three-Phase)31/2 -> Mux19/2  "Q(Wind)"
  PLL (3ph)4/2 -> Terminator4/1
  Sum4/1 -> Gain30/1
  From125/1 -> Sequence Analyzer17/1, PLL (3ph)4/1
  Mux19/1 -> Gain26/1  "PQ_Wind"
  From117/1 -> Power Measurement (Three-Phase)32/1
  Gain28/1 -> Mux21/2  "Q(grid)"
  Power Measurement (Three-Phase)33/1 -> Mux13/1  "P(BESS)"
  Mux20/1 -> Scope20/7
  Power Measurement (Three-Phase)30/2 -> Mux20/2  "Q(Gen)"
  From135/1 -> Power Measurement (Three-Phase)33/1
  PLL (3ph)4/1 -> Scope20/1
  From124/1 -> Power Measurement (Three-Phase)31/2
  Gain32/1 -> Mux21/1  "P(grid)"
  From122/1 -> Power Measurement (Three-Phase)32/2
  From123/1 -> Power Measurement (Three-Phase)31/1
  From133/1 -> Power Measurement (Three-Phase)22/1
  Power Measurement (Three-Phase)22/1 -> Sum4/2  "P(Grid)"
  Power Measurement (Three-Phase)32/2 -> Mux18/2  "Q(PV)"
  Mux12/1 -> Scope20/3
  From134/1 -> Power Measurement (Three-Phase)22/2
  From126/1 -> Power Measurement (Three-Phase)30/1
  Power Measurement (Three-Phase)34/1 -> Sum4/1  "P(Grid)"
  Gain30/1 -> Scope20/9  "PQ_load"
  From107/1 -> Power Measurement (Three-Phase)33/2
  Gain26/1 -> Scope20/6
  Mux21/1 -> Scope20/8
  From132/1 -> Power Measurement (Three-Phase)34/2
  From129/1 -> Power Measurement (Three-Phase)29/2
  Power Measurement (Three-Phase)33/2 -> Mux13/2  "Q(BESS)"
  Gain33/1 -> Scope20/2
  Mux13/1 -> Scope20/4
  Mux18/1 -> Scope20/5
  connections:
  Three-Phase Breaker4/LConn3 -- B13/RConn1 -- Three-Phase Breaker4/LConn2 -- B14/RConn1 -- B15/RConn1 -- B4/RConn1 -- B16/RConn1 -- B1/LConn1 -- B9/RConn1 -- Three-Phase Breaker4/LConn1
  B15/RConn2 -- B14/RConn2 -- B13/RConn2 -- B4/RConn2 -- B9/RConn2 -- B1/LConn2 -- B16/RConn2
  B9/RConn3 -- B15/RConn3 -- B14/RConn3 -- B13/RConn3 -- B16/RConn3 -- B1/LConn3 -- B4/RConn3
  B9/LConn3 -- FC_BESS/LConn3
  FC_BESS/LConn1 -- B9/LConn1
  B9/LConn2 -- FC_BESS/LConn2
  B4/LConn1 -- FC_PV_FirstSolar/LConn1
  B4/LConn2 -- FC_PV_FirstSolar/LConn2
  B4/LConn3 -- FC_PV_FirstSolar/LConn3
  B2/LConn3 -- Three-Phase Breaker/LConn3
  B2/LConn2 -- Three-Phase Breaker/LConn2
  B2/LConn1 -- Three-Phase Breaker/LConn1
  B3/RConn1 -- Transformer 1-MVA 13.2-kV/400-V1/RConn3
  B3/RConn3 -- Transformer 1-MVA 13.2-kV/400-V1/RConn1
  Transformer 1-MVA 13.2-kV/400-V1/LConn2 -- B5/LConn2
  Transformer 1-MVA 13.2-kV/400-V1/LConn1 -- B5/LConn3
  B3/RConn2 -- Transformer 1-MVA 13.2-kV/400-V1/RConn2
  Transformer 1-MVA 13.2-kV/400-V1/LConn3 -- B5/LConn1
  B5/RConn1 -- 10 km line2/RConn3 -- 10 km line1/LConn3
  B5/RConn2 -- 10 km line2/RConn2 -- 10 km line1/LConn2
  B5/RConn3 -- 10 km line2/RConn1 -- 10 km line1/LConn1
  B7/RConn1 -- Three-Phase Breaker2/RConn1
  B7/RConn3 -- Three-Phase Breaker2/RConn3
  B6/RConn3 -- Three-Phase Transformer (Two Windings)2/RConn3
  B6/RConn1 -- Three-Phase Transformer (Two Windings)2/RConn1
  B7/RConn2 -- Three-Phase Breaker2/RConn2
  B6/RConn2 -- Three-Phase Transformer (Two Windings)2/RConn2
  Three-Phase Breaker2/LConn1 -- B12/RConn1 -- B8/LConn1
  Three-Phase Breaker2/LConn2 -- B12/RConn2 -- B8/LConn2
  Three-Phase Breaker2/LConn3 -- B12/RConn3 -- B8/LConn3
  B8/RConn1 -- 10 km line2/LConn1
  B8/RConn2 -- 10 km line2/LConn2
  B8/RConn3 -- 10 km line2/LConn3
  Three-Phase Parallel RLC Load/LConn3 -- synchronous/RConn3 -- B6/LConn3
  B6/LConn2 -- synchronous/RConn2 -- Three-Phase Parallel RLC Load/LConn2
  Three-Phase Parallel RLC Load/LConn1 -- synchronous/RConn1 -- B6/LConn1
  B7/LConn1 -- Three-Phase Transformer (Two Windings)2/LConn1
  B7/LConn2 -- Three-Phase Transformer (Two Windings)2/LConn2
  B7/LConn3 -- Three-Phase Transformer (Two Windings)2/LConn3
  "Step load. 240 kW in paper "/LConn1 -- B10/LConn3
  "Step load. 240 kW in paper "/LConn3 -- B10/LConn1
  "Step load. 240 kW in paper "/LConn2 -- B10/LConn2
  Defferable Load (0-446.25 kW)/LConn3 -- SL/RConn1
  Defferable Load (0-446.25 kW)/LConn2 -- SL/RConn2
  Defferable Load (0-446.25 kW)/LConn1 -- SL/RConn3
  115 kV/13.2 kV 10 MVA Xcel Substation/RConn3 -- "Grounding Transformer "/LConn3 -- 10 km line/LConn3
  115 kV/13.2 kV 10 MVA Xcel Substation/RConn1 -- "Grounding Transformer "/LConn1 -- 10 km line/LConn1
  115 kV/13.2 kV 10 MVA Xcel Substation/RConn2 -- "Grounding Transformer "/LConn2 -- 10 km line/LConn2
  B3 (115 kV)/RConn2 -- 115 kV/13.2 kV 10 MVA Xcel Substation/LConn2
  "3.3ohms "/LConn1 -- "Grounding Transformer "/RConn1
  B3 (115 kV)/RConn3 -- 115 kV/13.2 kV 10 MVA Xcel Substation/LConn3
  "3.3ohms "/RConn1 -- Ground2/LConn1
  Ground1/LConn1 -- 115 kV/LConn1
  115 kV/RConn1 -- 2500 MVA X0/X1=3/LConn1
  B3 (115 kV)/LConn2 -- 2500 MVA X0/X1=3/RConn2
  115 kV/RConn3 -- 2500 MVA X0/X1=3/LConn3
  B3 (115 kV)/RConn1 -- 115 kV/13.2 kV 10 MVA Xcel Substation/LConn1
  B3 (115 kV)/LConn3 -- 2500 MVA X0/X1=3/RConn3
  115 kV/RConn2 -- 2500 MVA X0/X1=3/LConn2
  B3 (115 kV)/LConn1 -- 2500 MVA X0/X1=3/RConn1
  10 km line/RConn1 -- B2/RConn1
  10 km line/RConn2 -- B2/RConn2
  10 km line/RConn3 -- B2/RConn3
  B3/LConn1 -- Subsystem4/RConn3
  B3/LConn2 -- Subsystem4/RConn2
  Subsystem4/RConn1 -- B3/LConn3
  B11/LConn2 -- Crit load. 900kW in paper/LConn2
  B11/LConn1 -- Crit load. 900kW in paper/LConn3
  B11/LConn3 -- Crit load. 900kW in paper/LConn1
  Three-Phase Breaker1/RConn3 -- B10/RConn3
  Three-Phase Breaker1/RConn2 -- B10/RConn2
  Three-Phase Breaker1/RConn1 -- B10/RConn1
  Three-Phase Breaker3/RConn3 -- B11/RConn3
  Three-Phase Breaker3/RConn2 -- B11/RConn2
  Three-Phase Breaker3/RConn1 -- B11/RConn1
  B12/LConn1 -- Three-Phase Dynamic Load/LConn1
  B12/LConn2 -- Three-Phase Dynamic Load/LConn2
  B12/LConn3 -- Three-Phase Dynamic Load/LConn3
  Three-Phase Fault/LConn1 -- Three-Phase Breaker4/RConn1
  Three-Phase Breaker4/RConn3 -- Three-Phase Fault/LConn3
  Three-Phase Breaker4/RConn2 -- Three-Phase Fault/LConn2
  Load Flow Bus2/LConn1 -- 10 km line1/RConn1 -- B13/LConn1
  10 km line1/RConn2 -- B13/LConn2
  B13/LConn3 -- 10 km line1/RConn3
  B14/LConn1 -- Three-Phase Breaker1/LConn1
  B14/LConn2 -- Three-Phase Breaker1/LConn2
  B14/LConn3 -- Three-Phase Breaker1/LConn3
  B15/LConn1 -- Three-Phase Breaker3/LConn1
  B15/LConn2 -- Three-Phase Breaker3/LConn2
  B15/LConn3 -- Three-Phase Breaker3/LConn3
  Subsystem4/LConn1 -- Wind Turbine Type 4/LConn1
  Subsystem4/LConn2 -- Wind Turbine Type 4/LConn2
  Subsystem4/LConn3 -- Wind Turbine Type 4/LConn3
  B1/RConn1 -- Three-Phase Breaker/RConn1
  B1/RConn2 -- Three-Phase Breaker/RConn2
  B1/RConn3 -- Three-Phase Breaker/RConn3
  B16/LConn1 -- MODEL STABILIZER/LConn1
  B16/LConn3 -- MODEL STABILIZER/LConn3
  B16/LConn2 -- MODEL STABILIZER/LConn2
